simulink model "HDVSim_Hybrid_Truck_Platooning"  (R2018b)
settings: Solver=ode3  StartTime=0.0  StopTime=inf  FixedStep=sample_time  MaxStep=0.1  RelTol=1e-3  EnableMultiTasking=on
model workspace (MAT data in the model file):
  Anschaffungskosten = [3707764736; 2; 1; 1; 1; 1]
  Bat.SOC_start = 1
  Bat.Voltage = 800
  Bat.Useable_range = 0.8
  Bat.Charge_cycles = 3202.25561185
  Bat.Useable_capacity = 61.538
  Bat.Efficiency_power_electronics = 0.95
  Bat.Type = 2
  Driving_cycle = 18
  Eigenschaften = []
  Electric_Truck = 0
  Elektro_LKW = 0
  FuelCell.P_nom = 0
  Fueltype = 1
  Gewichte = [3707764736; 2; 1; 1; 2; 2]
  Hybrid_Truck = 0
  IZ12 = 3600
  Kraftstoff = 1
  M_el = 1000
  SOC_T_EM_completely_available = 0.5
  SOC_addition = 0.4
  SOC_el = 0.8
  SOC_target = 0.85
  Sailing_without_drag_torque = 0
  TCO = TCO
  TCO.Verhaeltnis_Anh_Lkw = [1 1]
  TCO.Kaufpreis = [89248 59191]
  TCO.Preisanstieg_Wiederbeschaffung = [3.5 3.5]
  TCO.Wiederbeschaffungsneupreis = [59774 54183]
  TCO.Restwert = [26774 0]
  TCO.CNG_Verbrauch = 0
  TCO.LNG_Verbrauch = 0
  TCO.Wasserstoffverbrauch = 0
  TCO.Reifenkosten_Satz = [2700 5008]
  TCO.Abschreibungswert = [73478 81874]
  TCO.Mautsatz = 0.135
  TCO.Tagesarbeitszeit = 8
  TCO.Sonstige_Arbeiten_Tag = 0.5
  TCO.Bruttostundenlohn_Fahrer = 13
  TCO.Einsatztage_Jahr = 240
  TCO.Jahresbruttolohn_Fahrer = 24960
  TCO.Personalfaktor = 1.3
  TCO.Jahresbruttolohn_FZG = 32448
  TCO.Sozialaufwendungen_Proz = 25.75
  TCO.Sozialaufwendungen_EUR = 8355
  TCO.Aushilfsfahrer = 0
  TCO.Spesen_Tag = 12
  TCO.Spesen_Jahr = 2880
  TCO.Fahrerkosten_Sonstige = 0
  TCO.Fahrpersonalkosten_Summe = 43683
  TCO.Dieselpreis = 0.95
  TCO.Dieselpreis_Fremd = 1
  TCO.Adbluepreis = 0.68
  TCO.CNGpreis = 0.88
  TCO.LNGpreis = 0.81
  TCO.Strompreis = 0.12
  TCO.Wasserstoffpreis = 9
  TCO.Verzinsung_Umlaufvermoegen = 8.4
  TCO.Verzinsung_Anlagevermoegen = 8.4
  TCO.Verwaltungskosten = 10.7
  TCO.Fahrtstrecke = 50.1189193262
  TCO.Anteil_Mautstrecke = 75
  TCO.Beladezeit_Gespann = 0.25
  TCO.Entladezeit_Gespann = 0.25
  TCO.Anteil_Leerfahrten = 0
  TCO.Durchschnittsgeschwindigkeit = 84.1549018536
  TCO.Tageslenkzeit = 4.08
  TCO.Jahresfahrleistung = [82404 82404]
  TCO.Nutzungsdauer = [6 12]
  TCO.Reifenfahrleistung = [140000 170000]
  TCO.Anteil_Eigentankung_Diesel = 75
  TCO.Schmierstoffverbauch = 1
  TCO.Adblueverbrauch = 4
  TCO.Afa_zeitabhaengig = [100 100]
  TCO.Afa_leistungsabhaengig = [0 0]
  TCO.Umlaufvermoegen = [6000 1400]
  TCO.Steuern = [556 373]
  TCO.Versicherung_Kfz = [6298 677]
  TCO.Versicherung_Transport = 1000
  TCO.Kommunikation = 600
  TCO.Reparaturen_Wartung_Pflege = [0.13 0.025]
  TCO.Abschreibung_zeitabh = [12246 6823]
  TCO.Umlaufvermoegen_verzinst = 622
  TCO.Anlagevermoegen_verzinst = [3748 2486]
  TCO.Versicherung = [7298 677]
  TCO.Summe_Fzg_Kosten = [25070 10359]
  TCO.Summe_fixe_Kosten = [68753 10359]
  TCO.Abschreibung_leistungsabh = [0 0]
  TCO.Reparaturkosten = [10713 2060]
  TCO.Reifenkosten = [1589 2428]
  TCO.Lebensdauer_Batteriepack = 0
  TCO.Anschaffungspreis_Akkupack = 0
  TCO.Verschleisskosten_Batteriepack = 0
  TCO.Summe_variable_Kosten = [12302 4488]
  TCO.Summe_fixe_variable_Kosten = [81055 14847]
  TCO.Gemeinkosten = 11491
  TCO.Mautkosten = 8343.405
  TCO.Gesamtkosten = 115736.405
  TCO.Ergebnis = table
  TCO.Ergebnis.data = {{[]; 19069; 622; 6234; 929; 7975; 600; 35429; 43683; 79112; []; 0; 0; 0; 12773; 0; 4017; 16790; []; 95902; 11491; 8343.405; 115736.405}, {[]; 0.231408669482; 0.00754817727295; 0.0756516673948; 0.0112737245765; 0.0967792825591; 0.00728119994175; 0.429942721227; 0.530107761759; 0.960050482986; []; 0; 0; 0; 0.155004611427; 0; 0.04874763361; 0.203752245037; []; 1.16380272802; 0.139447114218; 0.10125; 1.40449984224}, {[]; []; []; []; []; []; []; []; []; []; []; []; []; []; []; []; []; []; []; []; []; []; []}, {'#cccccc'; '#9DFF00'; '#CEFF00'; '#FFFF00'; '#FFDF00'; '#FFB900'; '#FF9200'; '#FF5D00'; '#FF7F7F'; '#FF2900'; '#cccccc'; '#00FF85'; '#00FFC6'; '#00FFF2'; '#00FFFF'; '#00DBFF'; '#00B3FF'; '#0088FF'; '#cccccc'; '#B100FF'; '#FF00FF'; '#FF00C0'; '#FF0070'}, [0; 1; 1; 1; 1; 1; 1; 0; 1; 0; 0; 1; 1; 1; 1; 1; 1; 0; 0; 0; 1; 1; 0]}
  TCO.Ergebnis.ndims = 2
  TCO.Ergebnis.nrows = 23
  TCO.Ergebnis.rownames = {'Zeitabh_Fzg_Kosten'; 'Abschreibung_zeitabh'; 'Umlaufvermoegen_verzinst'; 'Anlagevermoegen_verzinst'; 'Steuern'; 'Versicherung'; 'Kommunikation'; 'Summe_Fzg_Kosten'; 'Fahrpersonalkosten_Summe'; 'Summe_fixe_Kosten'; 'Leistungsabh_Fzg_Kosten'; 'Abschreibung_leistungsabh'; 'Kraftstoffkosten'; 'Adbluekosten'; 'Reparaturkosten'; 'Schmierstoffkosten'; 'Reifenkosten'; 'Summe_variable_Kosten'; 'Summe_Kosten'; 'Summe_fixe_variable_Kosten'; 'Gemeinkosten'; 'Mautkosten'; 'Gesamtkosten'}
  TCO.Ergebnis.nvars = 5
  TCO.Ergebnis.varnames = {'Euro_Jahr', 'Euro_km', 'Prozent', 'Cellcolor', 'Diagramm'}
  TCO.Ergebnis.props.CustomProps = struct()
  TCO.Ergebnis.props.VariableCustomProps = struct()
  TCO.Ergebnis.props.versionSavedFrom = 3
  TCO.Ergebnis.props.minCompatibleVersion = 1
  TCO.Ergebnis.props.incompatibilityMsg = ''
  TCO.Ergebnis.props.VersionSavedFrom = 3
  TCO.Ergebnis.props.Description = ''
  TCO.Ergebnis.props.DimensionNames = {'Row', 'Variables'}
  TCO.Ergebnis.props.UserData = []
  TCO.Ergebnis.props.VariableDescriptions = {}
  TCO.Ergebnis.props.VariableUnits = {}
  TCO.Ergebnis.props.VariableContinuity = {}
  TCO_Anhaenger = 1
  TCO_Trailer = 1
  T_distance_LPS_down = 250
  T_distance_LPS_up = 250
  VSim.Display = 3
  VSim.Opt = 0
  VSim.v_t = [0 0 0 0 0 0 1.65166299447 3.48693546103 5.32196202623 7.15649366725 8.99043956604 10.9164984764 14.0784276146 19.1118285963 24.3934691092 29.026743167 31.4408667289 30.4086481328 33.8215646226 37.2573263956 40.6862952223 44.1078751777 47.5214696449 50.9264939062 54.3223705164 57.7085257373 61.0843888586 64.4493705574 67.8028976245 71.1444114206 74.4733381735 77.7891152098 81.0911158753 84.3786820499 87.3671173407 86.464344428 86.4690301672 86.4747021938 86.4803197388 86.4858626831 86.4913275703 86.4967182207 86.5020271743]
  Vehicle = 'empty'
  WPT.Voltage = 0
  WPT.P_max = 120
  WPT.expansion = 0.42
  WPT.eta = 0.92
  WPT.SOC_target = 1
  WPT.SOC_electric_only = 1
  acquisition_costs = [3707764736; 2; 1; 1; 5; 5]
  addition_for_critical_slope = 0.01
  ambient.gravity = 9.80665
  ambient.air_density = 1.1883
  ambient.friction_coeff = 0.8
  auxiliary_consumers.onBattery = 0
  auxiliary_consumers.power = 3500
  auxiliary_consumers.coolingSystem = [2.07882285003 1.39429153551 1.17315152225 1.09571031996 1.06766795776 1.05740509167 1.05341861849 1.05184466719 1.05110543918 1.05094477446 1.05078585401 1.05075614757 ... (2400 elements, 2400x1)]
  critical_altitude_difference = 50
  cycle.stop_end = 5
  cycle.stop_start = 5
  cycle.speed_init = 0
  cycle.distance = [1 2 3 4 5 6 7 8 9 10 11 12 ... (50000 elements, 1x50000)]
  cycle.speed = [23.6111111111 23.6111111111 23.6111111111 23.6111111111 23.6111111111 23.6111111111 23.6111111111 23.6111111111 23.6111111111 23.6111111111 23.6111111111 23.6111111111 ... (50000 elements, 1x50000)]
  cycle.slope = [-0.005 -0.005 -0.005 -0.005 -0.005 -0.005 -0.005 -0.005 -0.005 -0.005 -0.005 -0.005 ... (50000 elements, 1x50000)]
  cycle.altitude = [0 0 0 0 0 0 0 0 0 0 0 0 ... (50000 elements, 1x50000)]
  cycle.delta12 = [5 5 5 5 5 5 5 5 5 5 5 5 ... (50000 elements, 1x50000)]
  cycle.delta23 = [5 5 5 5 5 5 5 5 5 5 5 5 ... (50000 elements, 1x50000)]
  cycle.stop_time = [0 0 0 0 0 0 0 0 0 0 0 0 ... (50000 elements, 1x50000)]
  dcycle = 18
  distance_1_PPC = 175
  distance_2_PPC = 200
  distance_PPC_altitude_difference = 10000
  driver.controller_proportional_gain = 230000
  driver.controller_integral_gain = 3000
  driver.slew_rate_throttle_in = 2
  driver.slew_rate_throttle_out = -2
  driver.slew_rate_brake_in = 2
  driver.slew_rate_brake_out = -2
  em.P_max = 130
  em.M_max = 1050
  em.n_max = 2000
  em.n_eck = 1182.29386297
  em.speed = [0 10 20 30 40 50 60 70 80 90 100 110 120 130 140 150 160 170 180 190 200 210 220 230 240 250 260 270 280 290 300 310 320 330 340 350 360 370 380 390 400 410 420 430 440 450 460 470 480 490 500 510 520 530 540 550 560 570 580 590 600 610 620 630 640 650 660 670 680 690 700 710 720 730 740 750 760 770 780 790 800 810 820 830 840 850 860 870 880 890 900 910 920 930 940 950 960 970 980 990 1000 1010 1020 1030 1040 1050 1060 1070 1080 1090 1100 1110 1120 1130 1140 1150 1160 1170 1180 1190 1200 1210 1220 1230 1240 1250 1260 1270 1280 1290 1300 1310 1320 1330 1340 1350 1360 1370 1380 1390 1400 1410 1420 1430 1440 1450 1460 1470 1480 1490 1500 1510 1520 1530 1540 1550 1560 1570 1580 1590 1600 1610 1620 1630 1640 1650 1660 1670 1680 1690 1700 1710 1720 1730 1740 1750 1760 1770 1780 1790 1800 1810 1820 1830 1840 1850 1860 1870 1880 1890 1900 1910 1920 1930 1940 1950 1960 1970 1980 1990 2000]
  em.trq = [1050 1050 1050 1050 1050 1050 1050 1050 1050 1050 1050 1050 1050 1050 1050 1050 1050 1050 1050 1050 1050 1050 1050 1050 1050 1050 1050 1050 1050 1050 1050 1050 1050 1050 1050 1050 1050 1050 1050 1050 1050 1050 1050 1050 1050 1050 1050 1050 1050 1050 1050 1050 1050 1050 1050 1050 1050 1050 1050 1050 1050 1050 1050 1050 1050 1050 1050 1050 1050 1050 1050 1050 1050 1050 1050 1050 1050 1050 1050 1050 1050 1050 1050 1050 1050 1050 1050 1050 1050 1050 1050 1050 1050 1050 1050 1050 1050 1050 1050 1050 1050 1050 1050 1050 1050 1050 1050 1050 1050 1050 1050 1050 1050 1050 1050 1050 1050 1050 1050 1043.20046733 1034.5071301 1025.95748439 1017.54799682 1009.27524888 1001.13593235 993.126844893 985.244885807 977.48705206 969.850434466 962.332214044 954.929658551 947.640119173 940.461027361 933.389891817 926.42429561 919.56189342 912.800408909 906.137632202 899.571417476 893.09968066 886.720397226 880.431600083 874.231377547 868.11787141 862.089275081 856.143831805 850.279832957 844.495616406 838.789564944 833.160104776 827.605704078 822.124871601 816.71615534 811.378141253 806.109452024 800.908745882 795.774715459 790.706086699 785.701617795 780.760098187 775.880347573 771.061214979 766.30157785 761.600341176 756.956436657 752.368821889 747.836479588 743.358416836 738.933664355 734.561275809 730.240327128 725.969915858 721.749160533 717.577200068 713.453193171 709.376317781 705.345770521 701.360766168 697.420537144 693.524333026 689.671420065 685.861080728 682.092613251 678.365331211 674.678563107 671.031651955 667.423954901 663.854842843 660.323700062 656.829923871 653.372924272 649.952123621 646.566956311 643.216868454 639.901317586 636.619772368 633.371712304 630.15662747 626.974018241 623.823395034 620.704278058]
  em.Type = 1
  em.fuel.co2_per_kwh = 504
  em.efficiency.characteristic_map = [0.001 0.001 0.001 0.001 0.001 0.001 0.001 0.001 0.001 0.001 0.001 0.001 ... (20301 elements, 101x201)]
  em.efficiency.speed = [0 10 20 30 40 50 60 70 80 90 100 110 120 130 140 150 160 170 180 190 200 210 220 230 240 250 260 270 280 290 300 310 320 330 340 350 360 370 380 390 400 410 420 430 440 450 460 470 480 490 500 510 520 530 540 550 560 570 580 590 600 610 620 630 640 650 660 670 680 690 700 710 720 730 740 750 760 770 780 790 800 810 820 830 840 850 860 870 880 890 900 910 920 930 940 950 960 970 980 990 1000 1010 1020 1030 1040 1050 1060 1070 1080 1090 1100 1110 1120 1130 1140 1150 1160 1170 1180 1190 1200 1210 1220 1230 1240 1250 1260 1270 1280 1290 1300 1310 1320 1330 1340 1350 1360 1370 1380 1390 1400 1410 1420 1430 1440 1450 1460 1470 1480 1490 1500 1510 1520 1530 1540 1550 1560 1570 1580 1590 1600 1610 1620 1630 1640 1650 1660 1670 1680 1690 1700 1710 1720 1730 1740 1750 1760 1770 1780 1790 1800 1810 1820 1830 1840 1850 1860 1870 1880 1890 1900 1910 1920 1930 1940 1950 1960 1970 1980 1990 2000]
  em.efficiency.torque = [0 10.5 21 31.5 42 52.5 63 73.5 84 94.5 105 115.5 126 136.5 147 157.5 168 178.5 189 199.5 210 220.5 231 241.5 252 262.5 273 283.5 294 304.5 315 325.5 336 346.5 357 367.5 378 388.5 399 409.5 420 430.5 441 451.5 462 472.5 483 493.5 504 514.5 525 535.5 546 556.5 567 577.5 588 598.5 609 619.5 630 640.5 651 661.5 672 682.5 693 703.5 714 724.5 735 745.5 756 766.5 777 787.5 798 808.5 819 829.5 840 850.5 861 871.5 882 892.5 903 913.5 924 934.5 945 955.5 966 976.5 987 997.5 1008 1018.5 1029 1039.5 1050]
  em_M_max = 1050
  engine.bsfc.be = [1463.81124945 1337.51367643 1219.93532707 1127.30261663 1034.66990619 942.037195751 849.40448531 756.771774869 664.139064428 571.506353987 478.873643547 386.240933106 ... (45451 elements, 301x151)]
  engine.bsfc.trqorig = [0 10 20 30 40 50 60 70 80 90 100 110 120 130 140 150 160 170 180 190 200 210 220 230 240 250 260 270 280 290 300 310 320 330 340 350 360 370 380 390 400 410 420 430 440 450 460 470 480 490 500 510 520 530 540 550 560 570 580 590 600 610 620 630 640 650 660 670 680 690 700 710 720 730 740 750 760 770 780 790 800 810 820 830 840 850 860 870 880 890 900 910 920 930 940 950 960 970 980 990 1000 1010 1020 1030 1040 1050 1060 1070 1080 1090 1100 1110 1120 1130 1140 1150 1160 1170 1180 1190 1200 1210 1220 1230 1240 1250 1260 1270 1280 1290 1300 1310 1320 1330 1340 1350 1360 1370 1380 1390 1400 1410 1420 1430 1440 1450 1460 1470 1480 1490 1500 1510 1520 1530 1540 1550 1560 1570 1580 1590 1600 1610 1620 1630 1640 1650 1660 1670 1680 1690 1700 1710 1720 1730 1740 1750 1760 1770 1780 1790 1800 1810 1820 1830 1840 1850 1860 1870 1880 1890 1900 1910 1920 1930 1940 1950 1960 1970 1980 1990 2000 2010 2020 2030 2040 2050 2060 2070 2080 2090 2100 2110 2120 2130 2140 2150 2160 2170 2180 2190 2200 2210 2220 2230 2240 2250 2260 2270 2280 2290 2300 2310 2320 2330 2340 2350 2360 2370 2380 2390 2400 2410 2420 2430 2440 2450 2460 2470 2480 2490 2500 2510 2520 2530 2540 2550 2560 2570 2580 2590 2600 2610 2620 2630 2640 2650 2660 2670 2680 2690 2700 2710 2720 2730 2740 2750 2760 2770 2780 2790 2800 2810 2820 2830 2840 2850 2860 2870 2880 2890 2900 2910 2920 2930 2940 2950 2960 2970 2980 2990 3000]
  engine.bsfc.speed = [600 610 620 630 640 650 660 670 680 690 700 710 720 730 740 750 760 770 780 790 800 810 820 830 840 850 860 870 880 890 900 910 920 930 940 950 960 970 980 990 1000 1010 1020 1030 1040 1050 1060 1070 1080 1090 1100 1110 1120 1130 1140 1150 1160 1170 1180 1190 1200 1210 1220 1230 1240 1250 1260 1270 1280 1290 1300 1310 1320 1330 1340 1350 1360 1370 1380 1390 1400 1410 1420 1430 1440 1450 1460 1470 1480 1490 1500 1510 1520 1530 1540 1550 1560 1570 1580 1590 1600 1610 1620 1630 1640 1650 1660 1670 1680 1690 1700 1710 1720 1730 1740 1750 1760 1770 1780 1790 1800 1810 1820 1830 1840 1850 1860 1870 1880 1890 1900 1910 1920 1930 1940 1950 1960 1970 1980 1990 2000 2010 2020 2030 2040 2050 2060 2070 2080 2090 2100]
  engine.bsfc.M_be_min_orig = [1000 1040 1080 1120 1130 1140 1150 1160 1170 1180 1190 1200 1480 1520 1560 1600 1640 1680 1720 1760 1800 1840 1880 1920 1960 2000 2040 2080 2120 2160 2200 2220 2240 2240 2240 2240 2230 2230 2140 2130 2130 2130 2130 2130 2130 2130 2130 2030 1840 1840 1830 1830 1830 1830 1830 1830 1830 1830 1830 1730 1730 1730 1730 1730 1720 1720 1720 1720 1720 1720 1720 1720 1720 1720 1720 1720 1720 1720 1720 1720 1710 1720 1710 1710 1710 1620 1620 1620 1620 1620 1620 1630 1640 1640 1650 1660 1670 1680 1690 1700 1710 1710 1710 1710 1710 1710 1710 1710 1710 1710 1900 1890 1890 1890 1890 1890 1890 1890 1880 1870 1860 1840 1830 1820 1810 1800 1780 1770 1760 1750 1740 1720 1710 1700 1690 1680 1660 1650 1640 1630 1620 0 0 0 0 0 0 0 0 0 0]
  engine.bsfc.trq = [0 10 20 30 40 50 60 70 80 90 100 110 120 130 140 150 160 170 180 190 200 210 220 230 240 250 260 270 280 290 300 310 320 330 340 350 360 370 380 390 400 410 420 430 440 450 460 470 480 490 500 510 520 530 540 550 560 570 580 590 600 610 620 630 640 650 660 670 680 690 700 710 720 730 740 750 760 770 780 790 800 810 820 830 840 850 860 870 880 890 900 910 920 930 940 950 960 970 980 990 1000 1010 1020 1030 1040 1050 1060 1070 1080 1090 1100 1110 1120 1130 1140 1150 1160 1170 1180 1190 1200 1210 1220 1230 1240 1250 1260 1270 1280 1290 1300 1310 1320 1330 1340 1350 1360 1370 1380 1390 1400 1410 1420 1430 1440 1450 1460 1470 1480 1490 1500 1510 1520 1530 1540 1550 1560 1570 1580 1590 1600 1610 1620 1630 1640 1650 1660 1670 1680 1690 1700 1710 1720 1730 1740 1750 1760 1770 1780 1790 1800 1810 1820 1830 1840 1850 1860 1870 1880 1890 1900 1910 1920 1930 1940 1950 1960 1970 1980 1990 2000 2010 2020 2030 2040 2050 2060 2070 2080 2090 2100 2110 2120 2130 2140 2150 2160 2170 2180 2190 2200 2210 2220 2230 2240 2250 2260 2270 2280 2290 2300 2310 2320 2330 2340 2350 2360 2370 2380 2390 2400 2410 2420 2430 2440 2450 2460 2470 2480 2490 2500 2510 2520 2530 2540 2550 2560 2570 2580 2590 2600 2610 2620 2630 2640 2650 2660 2670 2680 2690 2700 2710 2720 2730 2740 2750 2760 2770 2780 2790 2800 2810 2820 2830 2840 2850 2860 2870 2880 2890 2900 2910 2920 2930 2940 2950 2960 2970 2980 2990 3000]
  engine.bsfc.M_be_min = [1000 1040 1080 1120 1130 1140 1150 1160 1170 1180 1190 1200 1480 1520 1560 1600 1640 1680 1720 1760 1800 1840 1880 1920 1960 2000 2040 2080 2120 2160 2200 2220 2240 2240 2240 2240 2230 2230 2140 2130 2130 2130 2130 2130 2130 2130 2130 2030 1840 1840 1830 1830 1830 1830 1830 1830 1830 1830 1830 1730 1730 1730 1730 1730 1720 1720 1720 1720 1720 1720 1720 1720 1720 1720 1720 1720 1720 1720 1720 1720 1710 1720 1710 1710 1710 1620 1620 1620 1620 1620 1620 1630 1640 1640 1650 1660 1670 1680 1690 1700 1710 1710 1710 1710 1710 1710 1710 1710 1710 1710 1900 1890 1890 1890 1890 1890 1890 1890 1880 1870 1860 1840 1830 1820 1810 1800 1780 1770 1760 1750 1740 1720 1710 1700 1690 1680 1660 1650 1640 1630 1620 0 0 0 0 0 0 0 0 0 0]
  engine.full_load.speed = [600; 900; 1000; 1350; 2000; 2001; 2100]
  engine.full_load.trqorig = [1000; 2200; 2400; 2400; 1620; 0; 0]
  engine.full_load.trq = [1000; 2200; 2400; 2400; 1620; 0; 0]
  engine.full_load.power = [62.8318530718; 207.345115137; 251.327412287; 339.292006588; 339.292006588; 0; 0]
  engine.number = 1
  engine.M_max_original = 2400
  engine.M_max = 2400
  engine.scale_factor = 1
  engine.fuel.density = 830
  engine.fuel.co2_per_litre = 2.62
  engine.fuel.heat_of_combustion = 42500
  engine.fuel.LHV = 35.8
  engine.speed_min = 600
  engine.speed_max = 2100
  engine.idle_fuel_consumption = 1.5
  engine.drag_torque.trq = [0 -65.6 -98.9 -123.3 -134.32 -156.04 -176.72 -217.28 -234.63 -256.02 -273.98 -301.74 -324 -353.92 -376.32 -421.26 -450]
  engine.drag_torque.speed = [0 450 600 700 800 1000 1200 1500 1600 1700 1800 1900 2000 2100 2200 2300 2400]
  engine.rated_power = 323619.35891
  engine.shift_parameter.n_lo = 1000
  engine.shift_parameter.n_pref = 1200
  engine.shift_parameter.n1 = 600
  engine.shift_parameter.n2 = 800
  engine.shift_parameter.n3 = 1100
  engine.shift_parameter.n4 = 600
  engine.shift_parameter.n5 = 1200
  engine.shift_parameter.n6 = 2100
  engine.shift_parameter.M_max = 2400
  final_drive.ratio = 10
  final_drive.trq_eff = 0.98
  ifElectric = 1
  ifOptimized = 0
  look_ahead_PPC = 250
  max_distance = 50000
  name = 'Verbrauchssimulation_Hybrid_LKW_Platooning'
  propertie = [3707764736; 2; 1; 1; 6; 6]
  prospective_cruise_control = 0
  sample_time = 0.1
  tank.v_diesel = 500
  tank.v_cng = 0
  tank.v_lng = 0
  tank.m_h2 = 0
  tires.radius = 0.4465
  tires.roll_drag_coeff.total = 0.0043
  transmission.init_gear = 1
  transmission.shift_time = 1
  transmission.ratios = [1 1]
  transmission.trq_eff = [0.99 0.99]
  transmission.lamda = [1.0130058518 1.0130058518]
  transmission.z = 1
  v_PPC_delta = 2.77777777778
  v_max_electrical_drive_only = 13.8888888889
  vehicle.long_truck = 0
  vehicle.payload = 19300
  vehicle.frontal_area = 10.2
  vehicle.air_drag_coeff = [0.527  0.527  0.527  0.527  0.527  0.527  0.527  0.527  0.527  0.527; 0.527  0.527  0.527  0.527  0.527  0.527  0.527  0.527  0.527  0.527; 0.527  0.527  0.527  0.527  0.527  0.527  0.527  0.527  0.527  0.527; 0.527  0.527  0.527  0.527  0.527  0.527  0.527  0.527  0.527  0.527; 0.527  0.527  0.527  0.527  0.527  0.527  0.527  0.527  0.527  0.527; 0.527  0.527  0.527  0.527  0.527  0.527  0.527  0.527  0.527  0.527; 0.527  0.527  0.527  0.527  0.527  0.527  0.527  0.527  0.527  0.527; 0.527  0.527  0.527  0.527  0.527  0.527  0.527  0.527  0.527  0.527; 0.527  0.527  0.527  0.527  0.527  0.527  0.527  0.527  0.527  0.527; 0.527  0.527  0.527  0.527  0.527  0.527  0.527  0.527  0.527  0.527]
  vehicle.Fx_max = 90221.18
  vehicle.F_brake_max = 309890.14
  vehicle.mass = 12632.5464604
  vehicle_F_brake_max = 309890.14
  weights = weights
  weights.m_Engine = 1122.29
  weights.m_Gearbox = 125
  weights.m_Retarder = 82
  weights.m_tank_system = 51.6564603608
  weights.m_Fuel = 425
  weights.m_Exhaust = 203.4
  weights.m_Trailer = 5400
  weights.m_Total = 7232.54646036
  weights.m_Base = 5223.2
  weights.max_Payload = 27367.4535396
  weights.m_Max = 40000
  x = 1
values from neighbouring files (symbols this model uses):
  transmission = Transmission_gearing(1, 1, false, false, final_drive.ratio)    [Parameterizing.m]
undefined symbols (not defined in the file or in its folder): Ion, Lithium
libraries: simulink x23, powerlib x2, electricdrivelib x1
(part 1 of 3)
settings Model: Creator=Alexander Suessmann  LastModifiedBy=ga73rep
settings DataIOCC: SaveFormat=Array  SaveOutput=off  SignalLogging=off  DSMLogging=off  SignalLoggingName=datalog
settings OptimizationCC: DefaultParameterBehavior=Inlined  ExpressionDepthLimit=2147483647  InitFltsAndDblsToZero=on  LifeSpan=inf
settings DebuggingCC: UnderspecifiedInitializationDetection=Classic  MergeDetectMultiDrivingBlocksExec=none  SolverPrmCheckMsg=warning  MultiTaskDSMMsg=warning  MultiTaskCondExecSysMsg=none  FcnCallInpInsideContextMsg=warning  AllowSymbolicDim=off  StateNameClashWarn=warning  SFUnusedDataAndEventsDiag=none  SFUnexpectedBacktrackingDiag=none  SFInvalidInputDataAccessInChartInitDiag=none  SFNoUnconditionalDefaultTransitionDiag=none  SFTransitionOutsideNaturalParentDiag=none  SFUnreachableExecutionPathDiag=none  SFUndirectedBroadcastEventsDiag=none  SFTransitionActionBeforeConditionDiag=none  SFExecutionAtInitializationDiag=none
settings HardwareCC: ProdBitPerPointer=32  ProdBitPerSizeT=32  ProdBitPerPtrDiffT=32  ProdLargestAtomicFloat=None  ProdIntDivRoundTo=Undefined  ProdEndianess=Unspecified  ProdWordSize=32  ProdHWDeviceType=32-bit Generic
settings ModelReferenceCC: PropagateSignalLabelsOutOfModel=off
settings SFSimCC: SimUseLocalCustomCode=off
settings RTWCC: RTWUseLocalCustomCode=off
settings CodeAppCC: StateflowObjectComments=on
settings GRTTargetCC: TargetLangStandard=C89/C90 (ANSI)  GeneratePreprocessorConditionals=Disable all  CombineOutputUpdateFcns=off  GRTInterface=on
settings ConfigComp: CovMetricSettings=dw  CovHtmlReporting=on  CovSaveCumulativeToWorkspaceVar=on  CovSaveSingleToWorkspaceVar=on  CovExternalEMLEnable=off  CovSFcnEnable=off
settings SimscapeCC: SimscapeNormalizeSystem=off

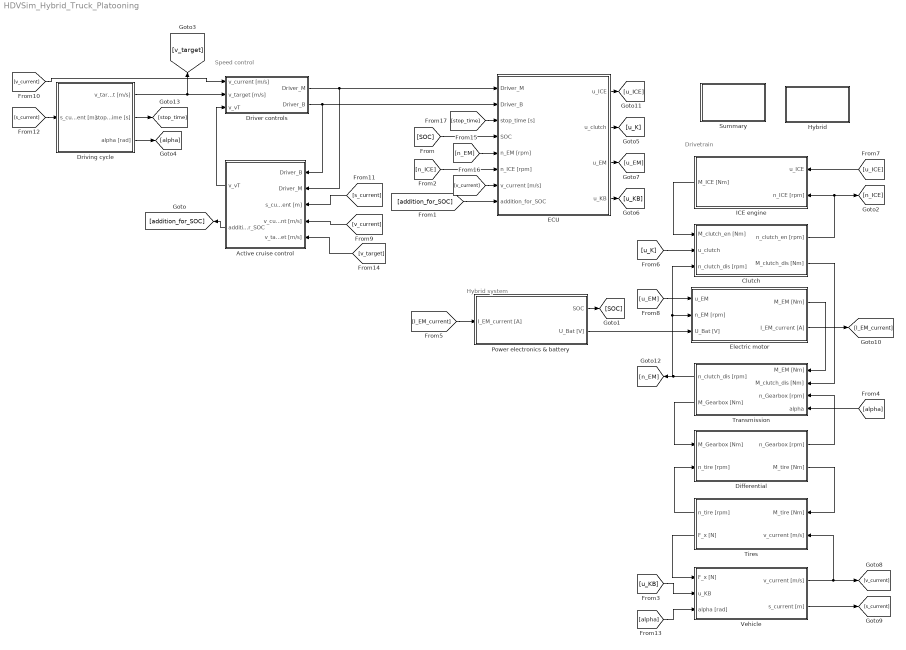
== system HDVSim_Hybrid_Truck_Platooning ==
  note: Hybrid system
  note: Speed control
  note: Drivetrain
  Active cruise control : Subsystem
  Clutch : Subsystem
  Differential : Subsystem
  Driver controls : Subsystem
  Driving cycle : Subsystem
  ECU : Subsystem
  Electric motor : Subsystem
  Hybrid : Subsystem
  ICE engine : Subsystem
  Power electronics & battery : Subsystem
  Summary : Subsystem
  Tires : Subsystem
  Transmission : Subsystem
  Vehicle : Subsystem
  wires:
  ICE engine/1(M_ICE [Nm]) -> Clutch/1(M_clutch_en [Nm])
  Transmission/1(n_clutch_dis [rpm]) -> Clutch/3(n_clutch_dis [rpm]), Electric motor/2(n_EM [rpm]), [n_EM]
  Transmission/2(M_Gearbox [Nm]) -> Differential/1(M_Gearbox [Nm])
  Tires/1(n_tire [rpm]) -> Differential/2(n_tire [rpm])
  Clutch/1(n_clutch_en [rpm]) -> [n_ICE], ICE engine/2(n_ICE [rpm])
  Clutch/2(M_clutch_dis [Nm]) -> Transmission/2(M_clutch_dis [Nm])
  Differential/1(n_Gearbox [rpm]) -> Transmission/3(n_Gearbox [rpm])
  Differential/2(M_tire [Nm]) -> Tires/1(M_tire [Nm])
  Vehicle/1(v_current [m/s]) -> [v_current], Tires/2(v_current [m/s])
  Tires/2(F_x [N]) -> Vehicle/1(F_x [N])
  Driver controls/2(Driver_B) -> Active cruise control/1(Driver_B), ECU/2(Driver_B)
  Electric motor/1(M_EM [Nm]) -> Transmission/1(M_EM [Nm])
  Active cruise control/2(addition_for_SOC) -> [addition_for_SOC]
  [addition_for_SOC] -> ECU/8(addition_for_SOC)
  Power electronics & battery/1(SOC) -> [SOC]
  [SOC] -> ECU/4(SOC)
  [n_ICE] -> ECU/6(n_ICE [rpm])
  Driving cycle/1(v_target [m/s]) -> [v_target], Driver controls/2(v_target [m/s])
  [v_current] -> Driver controls/1(v_current [m/s])
  [s_current] -> Driving cycle/1(s_current [m])
  Driving cycle/3(alpha [rad]) -> [alpha]
  Active cruise control/1(v_vT) -> Driver controls/3(v_vT)
  Driver controls/1(Driver_M) -> Active cruise control/2(Driver_M), ECU/1(Driver_M)
  [s_current] -> Active cruise control/3(s_current [m])
  [v_current] -> Active cruise control/4(v_current [m/s])
  [v_target] -> Active cruise control/5(v_target [m/s])
  Power electronics & battery/2(U_Bat [V]) -> Electric motor/3(U_Bat [V])
  [u_EM] -> Electric motor/1(u_EM)
  ECU/2(u_clutch) -> [u_K]
  [u_K] -> Clutch/2(u_clutch)
  ECU/4(u_KB) -> [u_KB]
  [u_KB] -> Vehicle/2(u_KB)
  [alpha] -> Vehicle/3(alpha [rad])
  Vehicle/2(s_current [m]) -> [s_current]
  [alpha] -> Transmission/4(alpha)
  Electric motor/2(I_EM_current [A]) -> [I_EM_current]
  [I_EM_current] -> Power electronics & battery/1(I_EM_current [A])
  ECU/3(u_EM) -> [u_EM]
  ECU/1(u_ICE) -> [u_ICE]
  [u_ICE] -> ICE engine/1(u_ICE)
  [n_EM] -> ECU/5(n_EM [rpm])
  [v_current] -> ECU/7(v_current [m/s])
  Driving cycle/2(stop_time [s]) -> [stop_time]
  [stop_time] -> ECU/3(stop_time [s])

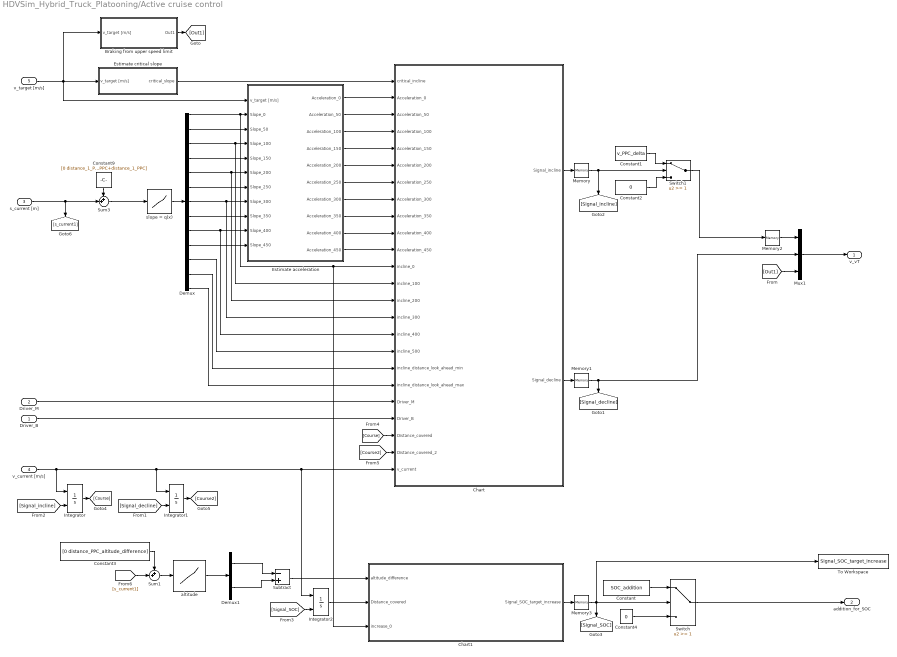
== system HDVSim_Hybrid_Truck_Platooning/Active cruise control ==
  Driver_B : Inport
  Driver_M : Inport  Port=2
  s_current [m] : Inport  Port=3
  v_current [m/s] : Inport  Port=4
  v_target [m/s] : Inport  Port=5
  Braking from upper speed limit : Subsystem
  Chart : Stateflow chart  TreatAsAtomicUnit=on
  Chart1 : Stateflow chart  TreatAsAtomicUnit=on
  Constant : Constant  Value=SOC_addition
  Constant1 : Constant  Value=v_PPC_delta
  Constant2 : Constant  Value=0
  Constant3 : Constant  Value=[0 distance_PPC_altitude_difference]
  Constant4 : Constant  Value=0
  Constant9 : Constant  Value=[0 distance_1_PPC/5 2*distance_1_PPC/5 3*distance_1_PPC/5 4*distance_1_PPC/5 distance_1_PPC 6*distance_1_PPC/5 7*distance_1_PPC/5 8*distance_1_PPC/5 9*distance_1_PPC/5 10*distance_1_PPC/5 look_ahead_PPC look_ahead_PPC+distance_1_PPC]
  Demux : Demux  Outputs=13
  Demux1 : Demux  Outputs=2
  Estimate acceleration : Subsystem
  Estimate critical slope : Subsystem
  Integrator : Integrator  ExternalReset=rising
  Integrator1 : Integrator  ExternalReset=rising
  Integrator2 : Integrator  ExternalReset=rising
  Memory{,1..3} (4 alike) : Memory
  Mux1 : Mux  Inputs=3
  Subtract : Sum  Inputs=-+
  Sum1 : Sum  Inputs=++|
  Sum3 : Sum  Inputs=++|
  Switch : Switch  Threshold=1
  Switch1 : Switch  Threshold=1
  To Workspace : ToWorkspace  VariableName=Signal_SOC_target_increase  SaveFormat=Structure With Time  SampleTime=-1
  altitude : Lookup_n-D  NumberOfTableDimensions=1  BreakpointsForDimension1=cycle.distance  Table=cycle.altitude  InterpMethod=Flat  RndMeth=Simplest  InputSameDT=on
  slope = q(x) : Lookup  InputValues=cycle.distance  Table=cycle.slope  LookUpMeth=Interpolation-Use End Values
  v_vT : Outport
  addition_for_SOC : Outport  Port=2
  wires:
  slope = q(x)/1 -> Demux/1
  Demux/1 -> Chart1/3(increase_0), Chart/12(incline_0), Estimate acceleration/2(Slope_0)
  Estimate critical slope/1(critical_slope) -> Chart/1(critical_incline)
  Chart/1(Signal_incline) -> Memory/1
  v_current [m/s]/1 -> Integrator/1, Integrator1/1, Chart/24(v_current), Integrator2/1
  Memory/1 -> [Signal_incline], Switch1/2
  Mux1/1 -> v_vT/1
  Constant9/1 -> Sum3/1
  Sum3/1 -> slope = q(x)/1
  Estimate acceleration/1(Acceleration_0) -> Chart/2(Acceleration_0)
  Estimate acceleration/2(Acceleration_50) -> Chart/3(Acceleration_50)
  Estimate acceleration/3(Acceleration_100) -> Chart/4(Acceleration_100)
  Estimate acceleration/4(Acceleration_150) -> Chart/5(Acceleration_150)
  Estimate acceleration/5(Acceleration_200) -> Chart/6(Acceleration_200)
  Estimate acceleration/6(Acceleration_250) -> Chart/7(Acceleration_250)
  Estimate acceleration/7(Acceleration_300) -> Chart/8(Acceleration_300)
  Estimate acceleration/8(Acceleration_350) -> Chart/9(Acceleration_350)
  Chart/2(Signal_decline) -> Memory1/1
  Memory1/1 -> Mux1/2, [Signal_decline]
  Driver_B/1 -> Chart/21(Driver_B)
  Estimate acceleration/9(Acceleration_400) -> Chart/10(Acceleration_400)
  Estimate acceleration/10(Acceleration_450) -> Chart/11(Acceleration_450)
  Driver_M/1 -> Chart/20(Driver_M)
  Demux/2 -> Estimate acceleration/3(Slope_50)
  Demux/3 -> Chart/13(incline_100), Estimate acceleration/4(Slope_100)
  Demux/4 -> Estimate acceleration/5(Slope_150)
  Demux/5 -> Chart/14(incline_200), Estimate acceleration/6(Slope_200)
  Demux/6 -> Estimate acceleration/7("Slope_250 ")
  Demux/7 -> Chart/15(incline_300), Estimate acceleration/8(Slope_300)
  Demux/8 -> Estimate acceleration/9(Slope_350)
  Demux/9 -> Chart/16(incline_400), Estimate acceleration/10(Slope_400)
  Demux/10 -> Estimate acceleration/11(Slope_450)
  Demux/12 -> Chart/18(incline_distance_look_ahead_min)
  Demux/13 -> Chart/19(incline_distance_look_ahead_max)
  v_target [m/s]/1 -> Braking from upper speed limit/1(v_target [m/s]), Estimate acceleration/1(v_target [m/s]), Estimate critical slope/1(v_target [m/s])
  Memory2/1 -> Mux1/1
  Constant1/1 -> Switch1/1
  Constant2/1 -> Switch1/3
  Demux/11 -> Chart/17(incline_500)
  Switch1/1 -> Memory2/1
  Constant3/1 -> Sum1/1
  s_current [m]/1 -> [s_current1], Sum3/2
  Sum1/1 -> altitude/1
  altitude/1 -> Demux1/1
  Demux1/2 -> Subtract/2
  Demux1/1 -> Subtract/1
  Subtract/1 -> Chart1/1(altitude_difference)
  Chart1/1(Signal_SOC_target_increase) -> Memory3/1
  Integrator2/1 -> Chart1/2(Distance_covered)
  Constant/1 -> Switch/1
  Constant4/1 -> Switch/3
  Switch/1 -> addition_for_SOC/1
  Memory3/1 -> Switch/2, To Workspace/1, [Signal_SOC]
  [Signal_decline] -> Integrator1/2
  Integrator1/1 -> [Course2]
  Integrator/1 -> [Course]
  [Signal_incline] -> Integrator/2
  [Course] -> Chart/22(Distance_covered)
  [Course2] -> Chart/23(Distance_covered_2)
  [Signal_SOC] -> Integrator2/2
  [s_current1] -> Sum1/2
  Braking from upper speed limit/1(Out1) -> [Out1]
  [Out1] -> Mux1/3

== system HDVSim_Hybrid_Truck_Platooning/Clutch ==
  note: Torque where clutch is disengaged
  note: Speed where clutch is engaged
  M_clutch_en [Nm] : Inport
  u_clutch : Inport  Port=2
  n_clutch_dis [rpm] : Inport  Port=3
  Compare To Zero : simulink/Logic and Bit Operations/Compare To Zero  relop===  OutDataTypeStr=boolean
  Constant : Constant  Value=0
  Idle engine speed : Constant  Value=engine.speed_min
  Logical Operator : Logic  AllPortsSameDT=off  OutDataTypeStr=boolean
  Lower engine speed : Saturate  UpperLimit=10000  LowerLimit=engine.speed_min  ZeroCross=off
  Null1 : Constant  Value=0
  Switch1 : Switch  Threshold=1
  Switch2 : Switch  Threshold=1
  Switch3 : Switch  Threshold=1
  n_clutch_en [rpm] : Outport
  M_clutch_dis [Nm] : Outport  Port=2
  wires:
  n_clutch_dis [rpm]/1 -> Lower engine speed/1
  Lower engine speed/1 -> Switch3/3
  Switch2/1 -> Switch1/3
  Null1/1 -> Switch2/1
  M_clutch_en [Nm]/1 -> Switch2/3
  [M_mot] -> Compare To Zero/1
  Compare To Zero/1 -> Logical Operator/1
  [ZKU] -> Logical Operator/2
  Logical Operator/1 -> Switch2/2
  Switch1/1 -> M_clutch_dis [Nm]/1
  Constant/1 -> Switch1/1
  Switch3/1 -> n_clutch_en [rpm]/1
  u_clutch/1 -> Switch1/2, Switch3/2
  Idle engine speed/1 -> Switch3/1

== system HDVSim_Hybrid_Truck_Platooning/Differential ==
  note: Effective wheel torque
  M_Gearbox [Nm] : Inport
  n_tire [rpm] : Inport  Port=2
  Differential efficiency : Constant  Value=final_drive.trq_eff
  Differential gear ratio : Constant  Value=final_drive.ratio
  M' = M*i*eta : Product  Inputs=***
  Product : Product  Inputs=/  RndMeth=Zero
  Switch : Switch  ZeroCross=off
  n' *i = n : Product  RndMeth=Zero
  n_Gearbox [rpm] : Outport
  M_tire [Nm] : Outport  Port=2
  tag scope: Eta_Axle_Drive=global
  wires:
  M_Gearbox [Nm]/1 -> M' = M*i*eta/1, Switch/2
  n_tire [rpm]/1 -> n' *i = n/2
  Differential gear ratio/1 -> n' *i = n/1, M' = M*i*eta/3
  n' *i = n/1 -> n_Gearbox [rpm]/1
  M' = M*i*eta/1 -> M_tire [Nm]/1
  Differential efficiency/1 -> Product/1, Switch/1
  Product/1 -> Switch/3
  Switch/1 -> [Eta_Axle_Drive], M' = M*i*eta/2

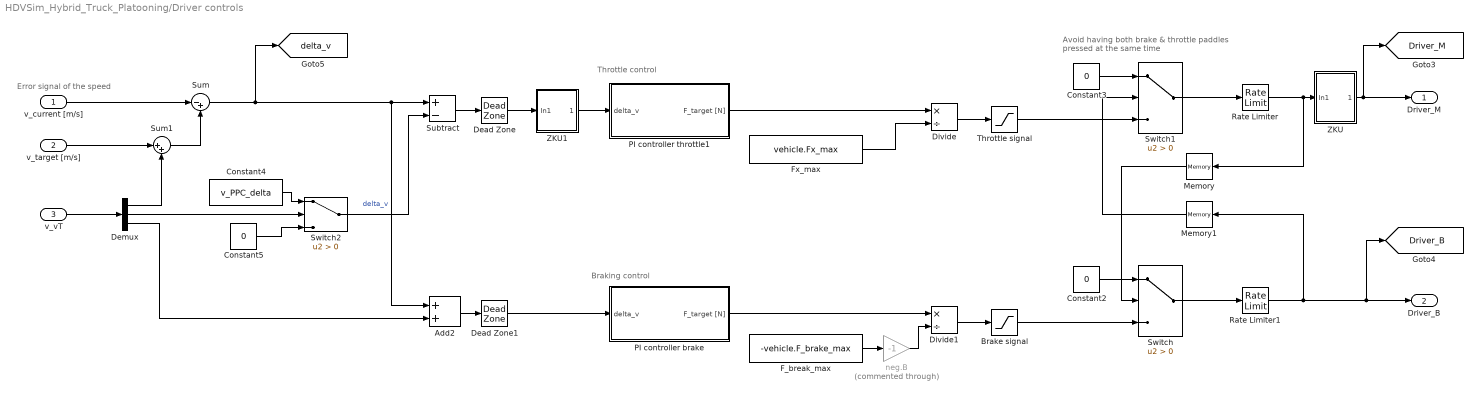
== system HDVSim_Hybrid_Truck_Platooning/Driver controls ==
  note: Avoid having both brake & throttle
      | paddles pressed at the same time
  note: Throttle control
  note: Braking control
  note: Error signal of the speed
  v_current [m/s] : Inport
  v_target [m/s] : Inport  Port=2
  v_vT : Inport  Port=3
  Add2 : Sum
  Brake signal : Saturate  UpperLimit=1  LowerLimit=0  ZeroCross=off
  Constant2 : Constant  Value=0
  Constant3 : Constant  Value=0
  Constant4 : Constant  Value=v_PPC_delta
  Constant5 : Constant  Value=0
  Dead Zone : DeadZone  LowerValue=-0.1/3.6  UpperValue=0.1/3.6  ZeroCross=off  SaturateOnIntegerOverflow=on
  Dead Zone1 : DeadZone  LowerValue=-0.1/3.6  UpperValue=0  ZeroCross=off  SaturateOnIntegerOverflow=on
  Demux : Demux  Outputs=3
  Divide : Product  Inputs=*/
  Divide1 : Product  Inputs=*/
  F_break_max : Constant  Value=-vehicle.F_brake_max
  Fx_max : Constant  Value=vehicle.Fx_max
  Memory : Memory
  Memory1 : Memory
  PI controller brake : Subsystem
  PI controller throttle1 : Subsystem
  Rate Limiter : RateLimiter  RisingSlewLimit=driver.slew_rate_throttle_in  FallingSlewLimit=driver.slew_rate_throttle_out  SampleTimeMode=inherited
  Rate Limiter1 : RateLimiter  RisingSlewLimit=driver.slew_rate_brake_in*100  FallingSlewLimit=driver.slew_rate_brake_out*100  SampleTimeMode=inherited
  Subtract : Sum  Inputs=+-
  Sum : Sum  Inputs=|-+
  Sum1 : Sum  Inputs=|++
  Switch : Switch  Criteria=u2 > Threshold
  Switch1 : Switch  Criteria=u2 > Threshold
  Switch2 : Switch  Criteria=u2 > Threshold
  Throttle signal : Saturate  UpperLimit=1  LowerLimit=0  ZeroCross=off
  ZKU : Subsystem
  ZKU1 : Subsystem
  neg.B : Gain  Commented=through  Gain=-1
  Driver_M : Outport
  Driver_B : Outport  Port=2
  tag scope: Driver_B=global, Driver_M=global, delta_v=global
  wires:
  Sum1/1 -> Sum/2
  v_current [m/s]/1 -> Sum/1
  Fx_max/1 -> Divide/2
  neg.B/1 -> Divide1/2
  Sum/1 -> [delta_v], Add2/1, Subtract/1  "delta_v"
  Divide1/1 -> Brake signal/1
  Divide/1 -> Throttle signal/1
  F_break_max/1 -> neg.B/1
  Switch/1 -> Rate Limiter1/1
  Brake signal/1 -> Switch/3
  Constant2/1 -> Switch/1
  Switch1/1 -> Rate Limiter/1
  Throttle signal/1 -> Switch1/3
  Rate Limiter1/1 -> Memory1/1, [Driver_B], Driver_B/1
  Rate Limiter/1 -> ZKU/1(In1), Memory/1
  Constant3/1 -> Switch1/1
  PI controller throttle1/1(F_target [N]) -> Divide/1
  Dead Zone/1 -> ZKU1/1(In1)
  Dead Zone1/1 -> PI controller brake/1(delta_v)
  PI controller brake/1(F_target [N]) -> Divide1/1
  ZKU/1(Out1) -> [Driver_M], Driver_M/1
  ZKU1/1(Out1) -> PI controller throttle1/1(delta_v)
  Memory/1 -> Switch/2
  Memory1/1 -> Switch1/2
  v_vT/1 -> Demux/1
  Switch2/1 -> Subtract/2
  Demux/2 -> Switch2/2
  Constant4/1 -> Switch2/1
  Constant5/1 -> Switch2/3
  Subtract/1 -> Dead Zone/1
  Demux/1 -> Sum1/2
  v_target [m/s]/1 -> Sum1/1
  Demux/3 -> Add2/2
  Add2/1 -> Dead Zone1/1

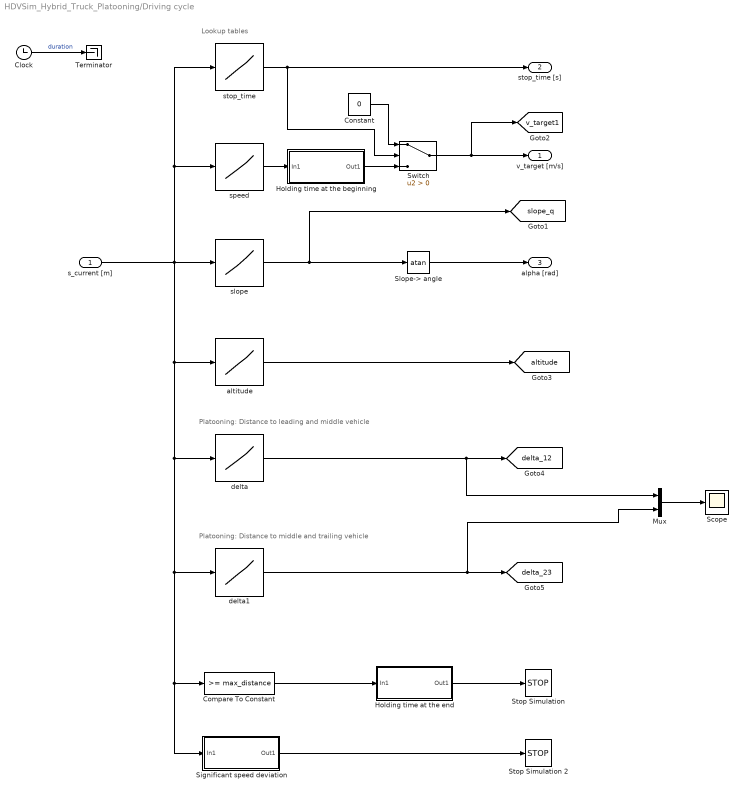
== system HDVSim_Hybrid_Truck_Platooning/Driving cycle ==
  note: Platooning: Distance to leading and middle vehicle
  note: Lookup tables
  note: Platooning: Distance to middle and trailing vehicle
  s_current [m] : Inport
  Clock : Clock
  Compare To Constant : simulink/Logic and Bit Operations/Compare To Constant  relop=>=  const=max_distance  OutDataTypeStr=boolean
  Constant : Constant  Value=0
  Holding time at the beginning : Subsystem
  Holding time at the end : Subsystem
  Mux : Mux  Inputs=2
  Scope : Scope
  Significant speed deviation : Subsystem
  Slope-> angle : Trigonometry  Operator=atan
  Stop Simulation : Stop
  Stop Simulation 2 : Stop
  Switch : Switch  Criteria=u2 > Threshold
  Terminator : Terminator
  altitude : Lookup_n-D  NumberOfTableDimensions=1  BreakpointsForDimension1=cycle.distance  Table=cycle.altitude  InterpMethod=Flat  RndMeth=Simplest  InputSameDT=on
  delta : Lookup_n-D  NumberOfTableDimensions=1  BreakpointsForDimension1=cycle.distance  BeginIndexSearchUsingPreviousIndexResult=on  Table=cycle.delta12  InterpMethod=Flat  RndMeth=Simplest  InputSameDT=on
  delta1 : Lookup_n-D  NumberOfTableDimensions=1  BreakpointsForDimension1=cycle.distance  BeginIndexSearchUsingPreviousIndexResult=on  Table=cycle.delta23  InterpMethod=Flat  RndMeth=Simplest  InputSameDT=on
  slope : Lookup_n-D  NumberOfTableDimensions=1  BreakpointsForDimension1=cycle.distance  Table=cycle.slope  InterpMethod=Flat  RndMeth=Simplest  InputSameDT=on
  speed : Lookup_n-D  NumberOfTableDimensions=1  BreakpointsForDimension1=cycle.distance  Table=cycle.speed  InterpMethod=Flat  RndMeth=Simplest  InputSameDT=on
  stop_time : Lookup_n-D  NumberOfTableDimensions=1  BreakpointsForDimension1=cycle.distance  Table=cycle.stop_time  InterpMethod=Flat  RndMeth=Simplest  InputSameDT=on
  v_target [m/s] : Outport
  stop_time [s] : Outport  Port=2
  alpha [rad] : Outport  Port=3
  tag scope: altitude=global, delta_12=global, delta_23=global, slope_q=global, v_target1=global
  wires:
  slope/1 -> Slope-> angle/1, [slope_q]
  Slope-> angle/1 -> alpha [rad]/1
  Compare To Constant/1 -> Holding time at the end/1(In1)
  Clock/1 -> Terminator/1  "duration"
  Switch/1 -> [v_target1], v_target [m/s]/1
  stop_time/1 -> stop_time [s]/1, Switch/2
  speed/1 -> Holding time at the beginning/1(In1)
  Holding time at the end/1(Out1) -> Stop Simulation/1
  Holding time at the beginning/1(Out1) -> Switch/3
  Constant/1 -> Switch/1
  altitude/1 -> [altitude]
  Significant speed deviation/1(Out1) -> Stop Simulation 2/1
  delta/1 -> Mux/1, [delta_12]
  s_current [m]/1 -> slope/1, delta/1, delta1/1, Significant speed deviation/1(In1), Compare To Constant/1, altitude/1, speed/1, stop_time/1
  delta1/1 -> Mux/2, [delta_23]
  Mux/1 -> Scope/1

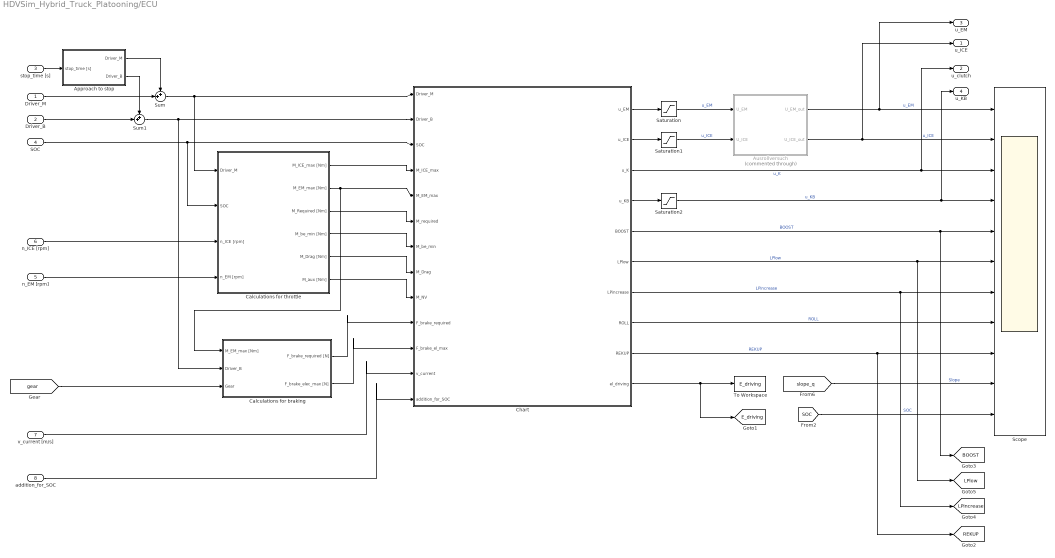
== system HDVSim_Hybrid_Truck_Platooning/ECU ==
  Driver_M : Inport
  Driver_B : Inport  Port=2
  stop_time [s] : Inport  Port=3
  SOC : Inport  Port=4
  n_EM [rpm] : Inport  Port=5
  n_ICE [rpm] : Inport  Port=6
  v_current [m/s] : Inport  Port=7
  addition_for_SOC : Inport  Port=8
  Approach to stop : Subsystem
  Ausrollversuch : Subsystem  Commented=through
  Calculations for braking : Subsystem
  Calculations for throttle : Subsystem
  Chart : Stateflow chart  TreatAsAtomicUnit=on
  Saturation : Saturate  UpperLimit=1  LowerLimit=-1
  Saturation1 : Saturate  UpperLimit=1  LowerLimit=0
  Saturation2 : Saturate  UpperLimit=1  LowerLimit=0
  Scope : Scope  NumInputPorts=11
  Sum : Sum  Inputs=++|
  Sum1 : Sum  Inputs=++|
  To Workspace : ToWorkspace  VariableName=E_driving  SampleTime=-1
      settings: Decimation=10
  u_ICE : Outport
  u_clutch : Outport  Port=2
  u_EM : Outport  Port=3
  u_KB : Outport  Port=4
  tag scope: BOOST=global, E_driving=global, LPincrease=global, LPlow=global, REKUP=global
  wires:
  Chart/1(u_EM) -> Saturation/1
  Chart/2(u_ICE) -> Saturation1/1
  Chart/4(u_KB) -> Saturation2/1
  Sum1/1 -> Calculations for braking/2(Driver_B), Chart/2(Driver_B)
  Sum/1 -> Calculations for throttle/1(Driver_M), Chart/1(Driver_M)
  Chart/3(u_K) -> u_clutch/1, Scope/3  "u_K"
  Calculations for braking/2(F_brake_elec_max [N]) -> Chart/11(F_brake_el_max)
  Calculations for braking/1(F_brake_required [N]) -> Chart/10(F_brake_required)
  SOC/1 -> Calculations for throttle/2(SOC), Chart/3(SOC)
  n_ICE [rpm]/1 -> Calculations for throttle/3(n_ICE [rpm])
  Calculations for throttle/1(M_ICE_max [Nm]) -> Chart/4(M_ICE_max)
  Calculations for throttle/3(M_Required [Nm]) -> Chart/6(M_required)
  Ausrollversuch/2(U_ICE_out) -> Scope/2, u_ICE/1  "u_ICE"
  Saturation2/1 -> u_KB/1, Scope/4  "u_KB"
  Calculations for throttle/5(M_Drag [Nm]) -> Chart/8(M_Drag)
  Calculations for throttle/4(M_be_min [Nm]) -> Chart/7(M_be_min)
  Chart/5(BOOST) -> [BOOST], Scope/5  "BOOST"
  Chart/8(ROLL) -> Scope/8  "ROLL"
  Chart/9(REKUP) -> [REKUP], Scope/9  "REKUP"
  Chart/7(LPincrease) -> [LPincrease], Scope/7  "LPincrease"
  [slope_q] -> Scope/10  "Slope"
  Calculations for throttle/6(M_aux [Nm]) -> Chart/9(M_NV)
  Chart/6(LPlow) -> [LPlow], Scope/6  "LPlow"
  Calculations for throttle/2(M_EM_max [Nm]) -> Calculations for braking/1(M_EM_max [Nm]), Chart/5(M_EM_max)
  [SOC] -> Scope/11  "SOC"
  Ausrollversuch/1(U_EM_out) -> u_EM/1, Scope/1  "u_EM"
  stop_time [s]/1 -> Approach to stop/1(stop_time [s])
  Approach to stop/2(Driver_B) -> Sum1/1
  Approach to stop/1(Driver_M) -> Sum/1
  Driver_M/1 -> Sum/2
  Driver_B/1 -> Sum1/2
  n_EM [rpm]/1 -> Calculations for throttle/4(n_EM [rpm])
  [gear] -> Calculations for braking/3(Gear)
  v_current [m/s]/1 -> Chart/12(v_current)
  Chart/10(el_driving) -> [E_driving], To Workspace/1
  addition_for_SOC/1 -> Chart/13(addition_for_SOC)
  Saturation1/1 -> Ausrollversuch/2(U_ICE)  "u_ICE"
  Saturation/1 -> Ausrollversuch/1(U_EM)  "u_EM"

== system HDVSim_Hybrid_Truck_Platooning/Electric motor ==
  note: Effective motor power
  note: Electric torque
  u_EM : Inport
  n_EM [rpm] : Inport  Port=2
  U_Bat [V] : Inport  Port=3
  Abs : Abs
  Abs1 : Abs
  Divide : Product  Inputs=*/
  Electric machine efficiency mapping : Lookup_n-D  BreakpointsForDimension1=em.efficiency.torque  BreakpointsForDimension2=em. efficiency.speed  Table=em.efficiency.characteristic_map  RndMeth=Simplest  InputSameDT=on
  Electric machine efficiency mapping2 : Lookup_n-D  BreakpointsForDimension1=em.efficiency.torque  BreakpointsForDimension2=em. efficiency.speed  Table=em.efficiency.characteristic_map  RndMeth=Simplest  InputSameDT=on
  Gain : Gain  Gain=2*pi/60
  Machine current demand : Subsystem
  Machine torque demand : Subsystem
  Math Function : Math  Operator=reciprocal  SaturateOnIntegerOverflow=on
  Product1 : Product
  Product2 : Product  Inputs=3
  Saturation : Saturate  UpperLimit=Bat.Useable_capacity / Bat.Useable_range*10  LowerLimit=-Bat.Useable_capacity / Bat.Useable_range*10
  Saturation1 : Saturate  UpperLimit=inf  LowerLimit=1
  Speed-torrque characteristics : Lookup_n-D  NumberOfTableDimensions=1  BreakpointsForDimension1=em.speed  Table=em.trq  ExtrapMethod=Clip  RndMeth=Simplest  InputSameDT=on
  Switch : Switch
  M_EM [Nm] : Outport
  I_EM_current [A] : Outport  Port=2
  tag scope: M_EM=global, n_EM=global, u_EM=global
  wires:
  Speed-torrque characteristics/1 -> Product1/1  "M_EM_max"
  u_EM/1 -> Product1/2, [u_EM]
  U_Bat [V]/1 -> Divide/2, Machine torque demand/4(U_Bat [V]), Machine current demand/4(U_Bat [V])  "U_Bat [V]"
  Machine current demand/1(I_target [A]) -> Saturation/1
  Saturation/1 -> Machine torque demand/2(I_current [A])
  Machine torque demand/1(M_EM [Nm]) -> Abs/1, Product2/3, [M_EM], M_EM [Nm]/1, Switch/2
  Gain/1 -> Product2/2
  Divide/1 -> I_EM_current [A]/1
  Math Function/1 -> Switch/1
  Electric machine efficiency mapping/1 -> Switch/3, Math Function/1  "Eta_EM"
  Switch/1 -> Product2/1
  Product2/1 -> Divide/1
  Abs/1 -> Electric machine efficiency mapping/1
  Product1/1 -> Machine current demand/2(M_EM_target [Nm]), Abs1/1  "M_EM_targetl"
  n_EM [rpm]/1 -> Electric machine efficiency mapping2/2, Saturation1/1, Electric machine efficiency mapping/2, Machine torque demand/1(n_EM [rpm]), Machine current demand/1("n_EM "), [n_EM], Speed-torrque characteristics/1  "n_EM [1/min]"
  Abs1/1 -> Electric machine efficiency mapping2/1
  Electric machine efficiency mapping2/1 -> Machine current demand/3(Eff_EM), Machine torque demand/3(Eff_EM)  "ETA_EM"
  Saturation1/1 -> Gain/1

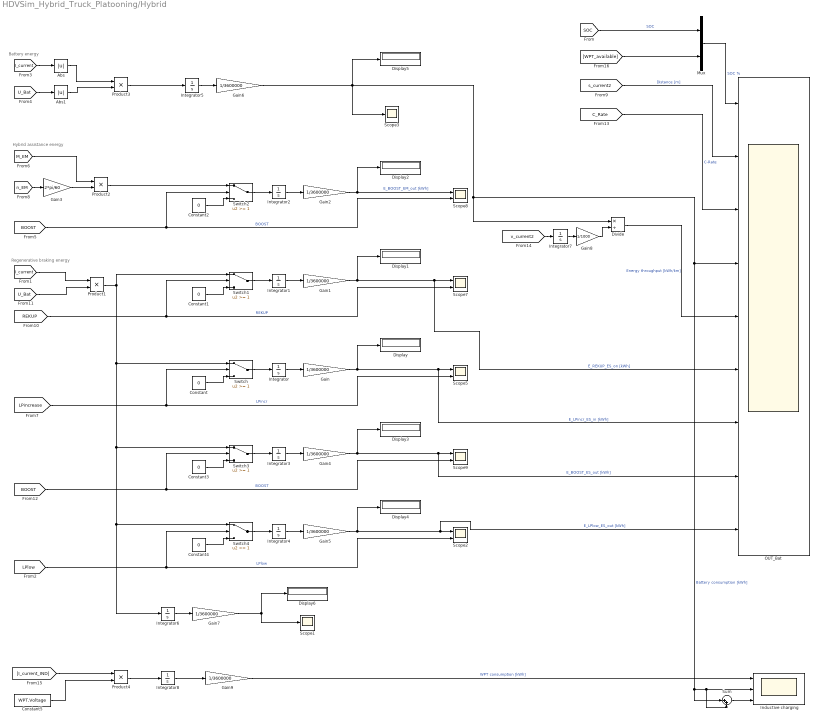
== system HDVSim_Hybrid_Truck_Platooning/Hybrid ==
  note: Regenerative braking energy
  note: Hybrid assistance energy
  note: Battery energy
  Abs : Abs
  Abs1 : Abs
  Constant{,1..4} (5 alike) : Constant  Value=0
  Constant5 : Constant  Value=WPT.Voltage
  Display{,1..6} (7 alike) : Display
  Divide : Product  Inputs=*/
  Gain{,1..2,4..7,9} (8 alike) : Gain  Gain=1/3600000
  Gain3 : Gain  Gain=2*pi/60
  Gain8 : Gain  Gain=1/1000
  Inductive charging : Scope  NumInputPorts=3
  Integrator{,1..6,8} (8 alike) : Integrator
  Integrator7 : Integrator  InitialCondition=0.00000001
  Mux : Mux  Inputs=2
  OUT_Bat : Scope  NumInputPorts=9
  Product{1..4} (4 alike) : Product
  Scope1 : Scope
  Scope{2,5,7..9} (5 alike) : Scope  NumInputPorts=2
  Scope3 : Scope
  Sum : Sum  Inputs=|++
  Switch{,1..4} (5 alike) : Switch  Threshold=1
  wires:
  Product1/1 -> Switch1/1, Switch/1, Switch3/1, Integrator6/1, Switch4/1
  Gain5/1 -> OUT_Bat/9, Scope2/1, Display4/1  "E_LPlow_ES_out [kWh]"
  Constant4/1 -> Switch4/3
  Integrator4/1 -> Gain5/1
  Switch4/1 -> Integrator4/1
  [LPlow] -> Scope2/2, Switch4/2  "LPlow"
  Gain4/1 -> OUT_Bat/8, Scope9/1, Display3/1  "E_BOOST_ES_out [kWh]"
  Constant3/1 -> Switch3/3
  Integrator3/1 -> Gain4/1
  Switch3/1 -> Integrator3/1
  [BOOST] -> Scope9/2, Switch3/2  "BOOST"
  Gain3/1 -> Product2/2
  [n_EM] -> Gain3/1
  Gain2/1 -> Scope8/1, Display2/1  "E_BOOST_EM_out [kWh]"
  Constant2/1 -> Switch2/3
  Integrator2/1 -> Gain2/1
  Switch2/1 -> Integrator2/1
  [BOOST] -> Scope8/2, Switch2/2  "BOOST"
  Product2/1 -> Switch2/1
  Gain1/1 -> OUT_Bat/6, Scope7/1, Display1/1  "E_REKUP_ES_on [kWh]"
  Constant1/1 -> Switch1/3
  Integrator1/1 -> Gain1/1
  Switch1/1 -> Integrator1/1
  [REKUP] -> Scope7/2, Switch1/2  "REKUP"
  [U_Bat] -> Product1/2
  [I_current] -> Product1/1
  Gain/1 -> OUT_Bat/7, Scope5/1, Display/1  "E_LPincr_ES_in [kWh]"
  Constant/1 -> Switch/3
  Integrator/1 -> Gain/1
  Switch/1 -> Integrator/1
  [LPincrease] -> Scope5/2, Switch/2  "LPincr"
  [M_EM] -> Product2/1
  [SOC] -> Mux/1  "SOC"
  Gain7/1 -> Display6/1, Scope1/1
  Integrator6/1 -> Gain7/1
  [U_Bat] -> Abs1/1
  [I_current] -> Abs/1
  Product3/1 -> Integrator5/1
  Integrator5/1 -> Gain6/1
  Abs/1 -> Product3/1
  Abs1/1 -> Product3/2
  [s_current2] -> OUT_Bat/2  "Distance [m]"
  [C_Rate] -> OUT_Bat/3  "C-Rate"
  Divide/1 -> OUT_Bat/5  "Energy throughput [kWh/km]"
  [v_current2] -> Integrator7/1
  Integrator7/1 -> Gain8/1
  Gain8/1 -> Divide/2
  Gain6/1 -> Scope3/1, Sum/1, Sum/2, Inductive charging/2, OUT_Bat/4, Divide/1, Display5/1  "Battery consumption [kWh]"
  [I_current_IND] -> Product4/1
  Constant5/1 -> Product4/2
  Product4/1 -> Integrator8/1
  Gain9/1 -> Inductive charging/1  "WPT consumption [kWh]"
  Integrator8/1 -> Gain9/1
  Sum/1 -> Inductive charging/3
  [WPT_available] -> Mux/2
  Mux/1 -> OUT_Bat/1  "SOC %"

== system HDVSim_Hybrid_Truck_Platooning/ICE engine ==
  note: Engine loading
  note: Consumption calculations
  u_ICE : Inport
  n_ICE [rpm] : Inport  Port=2
  Additional consumptions : Subsystem
  Consumption : Subsystem
  Drag torque : Lookup  InputValues=engine.drag_torque.speed  Table=engine.drag_torque.trq  LookUpMeth=Interpolation-Use End Values
  Full load curve : Lookup  InputValues=engine.full_load.speed  Table=engine.full_load.trq  LookUpMeth=Interpolation-Use End Values
  MinMax : MinMax  Inputs=2
  Product1 : Product
  Sum : Sum  Inputs=|+-
  Sum1 : Sum  Inputs=|++
  maximum engine torque due to tire slip : Subsystem
  M_ICE [Nm] : Outport
  tag scope: M_mot=global, n_mot=global
  wires:
  n_ICE [rpm]/1 -> Additional consumptions/2(n_clutch_en [rpm]), Consumption/2(n [rpm]), [n_mot], Drag torque/1, Full load curve/1
  Sum/1 -> Product1/2
  Product1/1 -> Sum1/1
  Drag torque/1 -> Sum1/2, Sum/2  "M_Drag"
  Additional consumptions/1(M_ICE_aftr_aux [Nm]) -> M_ICE [Nm]/1
  u_ICE/1 -> Product1/1
  Full load curve/1 -> MinMax/2  "M_ICE_max"
  Sum1/1 -> [M_mot], Additional consumptions/1(M_ICE_bfor_aux [Nm]), Consumption/1(M [Nm])
  maximum engine torque due to tire slip/1(M_mot_max_traction [Nm]) -> MinMax/1
  MinMax/1 -> Sum/1

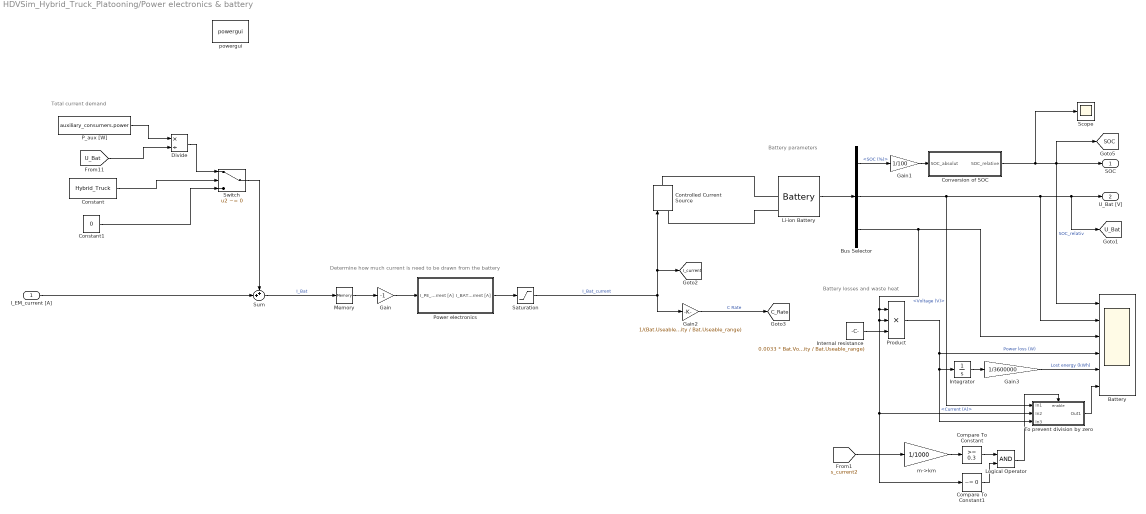
== system HDVSim_Hybrid_Truck_Platooning/Power electronics & battery ==
  note: Battery parameters
  note: Battery losses and waste heat
  note: Total current demand
  note: Determine how much current is need to be drawn from the battery
  I_EM_current [A] : Inport
  Battery : Scope  NumInputPorts=6
  Bus Selector : BusSelector  OutputSignals=SOC (%),Voltage (V),Current (A)
  Compare To Constant : simulink/Logic and Bit Operations/Compare To Constant  relop=>=  const=0.3  OutDataTypeStr=uint8  ZeroCross=off
  Compare To Constant1 : simulink/Logic and Bit Operations/Compare To Constant  relop=~=  const=0  OutDataTypeStr=uint8  ZeroCross=off
  Constant : Constant  Value=Hybrid_Truck
  Constant1 : Constant  Value=0
  Controlled Current Source : powerlib/Electrical Sources/Controlled Current Source  Initialize=off  Source_Type=DC  Amplitude=0  Phase=0  Frequency=0  Measurements=None
      settings: SourceProductName=Simscape Electrical
  Conversion of SOC : Subsystem
  Divide : Product  Inputs=*/
  Gain : Gain  Gain=-1
  Gain1 : Gain  Gain=1/100
  Gain2 : Gain  Gain=1/(Bat.Useable_capacity / Bat.Useable_range)
  Gain3 : Gain  Gain=1/3600000
  Integrator : Integrator
  Internal resistance : Constant  Value=0.0033 * Bat.Voltage / (Bat.Useable_capacity / Bat.Useable_range)
  Li-ion Battery : electricdrivelib/Extra Sources/Battery  BatType=Lithium-Ion  ShowTempParam=on  ThermalPreset=no  ShowAgeParam=off  NomV=Bat.Voltage  NomQ=Bat.Useable_capacity / Bat.Useable_range  SOC=(Bat.SOC_start *Bat.Useable_range+(0.5-Bat.Useable_range/2))* 100  Batt_Tr=30  PresetModel=off  MaxQ=Bat.Useable_capacity / Bat.Useable_range *8077/7500  MinV=487.5  FullV=Bat.Voltage * 1.178  Dis_rate=Bat.Useable_capacity / Bat.Useable_range * 1  R=0.0033 * Bat.Voltage / (Bat.Useable_capacity / Bat.Useable_range)  Normal_OP=Bat.Useable_capacity / Bat.Useable_range * 0.962  expZone="[Bat.Voltage*4339/4000     Bat.Useable_capacity / Bat.Useable_range/5]"  current=[5 25 50 250]  Units=Ampere-hour  Tci=20  NomT=20  T2=-30  MaxQ2=Bat.Useable_capacity / Bat.Useable_range *8077/7500  FullV2=Bat.Voltage * 1.178  Normal_OP2=487.5  expZone2="[Bat.Voltage*4339/4000     Bat.Useable_capacity / Bat.Useable_range/5]"  Rca=0.6  ti=1000  Dp=0  Neq0=0  Tsim=1e6  Ta1=25  Qeol=5.4*0.9  Reol=0.013333*1.2  Char_age=[2.3478, 3]  Dis_age=[2.3478, 10]  N1=1500  N2=10500  N3=1000  N4=1400  Ta2=45  N5=950
      settings: SourceProductName=Simscape Electrical
  Logical Operator : Logic  AllPortsSameDT=off  OutDataTypeStr=boolean
  Memory : Memory
  P_aux [W] : Constant  Value=auxiliary_consumers.power
  Power electronics : Subsystem
  Product : Product  Inputs=3
  Saturation : Saturate  UpperLimit=450  LowerLimit=-450
  Scope : Scope
  Sum : Sum  Inputs=++|
  Switch : Switch  Criteria=u2 ~= 0
  To prevent division by zero : Subsystem
  m->km : Gain  Gain=1/1000
  powergui : powerlib/powergui  Priority=1  SimulationMode=Discrete  SampleTime=sample_time  frequency=60  Iterations=50  frequencyindice=0  Pbase=100e6  ErrMax=1e-4  UnitsV=kV  UnitsW=MW  buscounter=0  FunctionMessages=off  echomessages=off  EnableUseOfTLC=off  CurrentSourceSwitches=off  DisableSnubberDevices=off  DisableRonSwitches=off  DisableVfSwitches=off  DisplayEquations=off  SolverType=Tustin  Interpol=off  ExternalGateDelay=off  methode=off  Ts=100  x0status=blocks  SPID=off  SwTol=0  HookPort=off  RestoreLinks=warning  ResistiveCurrentMeasurement=off  Frange=[0:2:500]  Ylog=off  Xlog=on  ShowGrid=off  save=off  variable=ZData  structure=0  ZoomFFT=off  StartTime=0.0  cycles=1  DisplayStyle=1  fundamental=60  FreqAxis=off  MaxFrequency=1000  frequencyindicesteady=1  RmsSteady=1  display=off
  SOC : Outport
  U_Bat [V] : Outport  Port=2
  tag scope: C_Rate=global, I_current=global, SOC=global, U_Bat=global
  wires:
  Li-ion Battery/1 -> Bus Selector/1
  Bus Selector/1 -> Gain1/1  "<SOC (%)>"
  Bus Selector/2 -> To prevent division by zero/1(In1), U_Bat [V]/1, [U_Bat], Battery/2  "<Voltage (V)>"
  Gain1/1 -> Conversion of SOC/1(SOC_absolut)
  Conversion of SOC/1(SOC_relative) -> Scope/1, SOC/1, [SOC], Battery/1  "SOC_relativ"
  I_EM_current [A]/1 -> Sum/2
  Saturation/1 -> Gain2/1, Controlled Current Source/1, [I_current]  "I_Bat_current"
  Gain2/1 -> [C_Rate]  "C Rate"
  [U_Bat] -> Divide/2
  P_aux [W]/1 -> Divide/1
  Constant/1 -> Switch/2
  Divide/1 -> Switch/1
  Constant1/1 -> Switch/3
  Switch/1 -> Sum/1
  Bus Selector/3 -> Product/1, Compare To Constant1/1, To prevent division by zero/2(In2), Product/2, Battery/3  "<Current (A)>"
  Internal resistance/1 -> Product/3
  Product/1 -> Battery/4, To prevent division by zero/3(In3), Integrator/1  "Power loss (W)"
  Integrator/1 -> Gain3/1
  Gain3/1 -> Battery/5  "Lost energy (kWh)"
  [s_current2] -> m->km/1
  m->km/1 -> Compare To Constant/1
  To prevent division by zero/1(Out1) -> Battery/6
  Compare To Constant/1 -> Logical Operator/1
  Compare To Constant1/1 -> Logical Operator/2
  Logical Operator/1 -> To prevent division by zero/Enable
  Gain/1 -> Power electronics/1(I_PE_current [A])
  Sum/1 -> Memory/1  "I_Bat"
  Memory/1 -> Gain/1
  Power electronics/1(I_BAT_current [A]) -> Saturation/1
  connections:
  Li-ion Battery/LConn1 -- Controlled Current Source/RConn1
  Li-ion Battery/LConn2 -- Controlled Current Source/LConn1

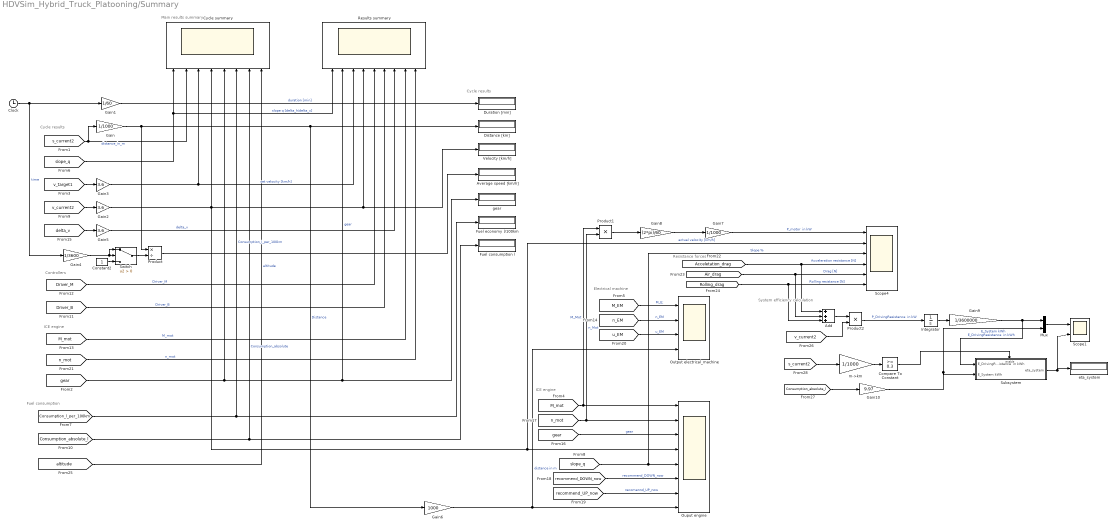
== system HDVSim_Hybrid_Truck_Platooning/Summary ==
  note: System efficiency calculation
  note: Resistance forces
  note: Electrical machine
  note: ICE engine
  note: Main results summary
  note: Cycle results
  note: Fuel consumption
  note: ICE engine
  note: Controllers
  note: Cycle results
  Add : Sum  Inputs=+++
  Average speed [km/h] : Display
  Clock : Clock
  Compare To Constant : simulink/Logic and Bit Operations/Compare To Constant  relop=>=  const=0.3  OutDataTypeStr=uint8  ZeroCross=off
  Constant2 : Constant
  Cycle summary : Scope  NumInputPorts=8
  Distance [km] : Display
  Duration [min] : Display
  Fuel consumption l : Display
  Fuel economy l/100km : Display
  Gain : Gain  Gain=1/1000
  Gain1 : Gain  Gain=1/60
  Gain10 : Gain  Gain=9.97
  Gain2 : Gain  Gain=3.6
  Gain3 : Gain  Gain=3.6
  Gain4 : Gain  Gain=1/3600
  Gain5 : Gain  Gain=3.6
  Gain6 : Gain  Gain=1000
  Gain7 : Gain  Gain=1/1000
  Gain8 : Gain  Gain=(2*pi)/60
  Gain9 : Gain  Gain=1/3600000
  Integrator : Integrator
  Mux : Mux  Inputs=2
  Ouput engine : Scope  NumInputPorts=8
  Output electrical_machine : Scope  NumInputPorts=4
  Product : Product  Inputs=*/  RndMeth=Zero
  Product1 : Product
  Product2 : Product
  Results summary : Scope  NumInputPorts=9
  Scope1 : Scope  NumInputPorts=2
  Scope4 : Scope  NumInputPorts=6
  Subsystem : Subsystem
  Switch : Switch  Criteria=u2 > Threshold
  Velocity [km/h] : Display
  eta_system : Display
  gear : Display
  m->km : Gain  Gain=1/1000
  wires:
  [v_current2] -> Gain2/1
  [s_current2] -> Cycle summary/2, Gain/1  "distance_in_m"
  Gain/1 -> Distance [km]/1, Gain6/1, Product/1  "Distance"
  Clock/1 -> Gain1/1, Gain4/1  "time"
  Gain1/1 -> Duration [min]/1  "duration [min]"
  Gain2/1 -> Ouput engine/4, Scope4/2, Results summary/4, Velocity [km/h]/1, Cycle summary/4  "actual velocity [km/h]"
  [gear] -> gear/1, Results summary/2, Cycle summary/5  "gear"
  [v_target1] -> Gain3/1
  [slope_q] -> Results summary/1, Cycle summary/1  "slope q [delta_h/delta_x]"
  [Consumption_l_per_100km] -> Cycle summary/6, Fuel economy l/100km/1  "Consumption_l_per_100km"
  Gain3/1 -> Cycle summary/3, Results summary/3  "set velocity [km/h]"
  Product/1 -> Average speed [km/h]/1
  [Consumption_absolute_l] -> Cycle summary/7, Fuel consumption l/1  "Consumption_absolute"
  [Driver_M] -> Results summary/5  "Driver_M"
  [Driver_B] -> Results summary/6  "Driver_B"
  [M_mot] -> Results summary/8  "M_mot"
  [delta_v] -> Gain5/1
  [M_mot] -> Ouput engine/1, Product1/1  "M_Mot"
  [n_mot] -> Ouput engine/2, Product1/2  "n_Mot"
  [gear] -> Ouput engine/3  "gear"
  [recommend_DOWN_now] -> Ouput engine/6  "recommend_DOWN_now"
  [recommend_UP_now] -> Ouput engine/7  "recomennd_UP_now"
  [slope_q] -> Ouput engine/5, Scope4/3  "Slope %"
  Gain5/1 -> Results summary/7  "delta_v"
  [n_mot] -> Results summary/9  "n_mot"
  [M_EM] -> Output electrical_machine/1  "M_E;"
  [n_EM] -> Output electrical_machine/2  "n_EM"
  [u_EM] -> Output electrical_machine/3  "u_EM"
  Product1/1 -> Gain8/1
  Gain7/1 -> Scope4/1  "P_motor  in kW"
  [Acceletation_drag] -> Add/1, Scope4/4  "Acceleration resistance [N]"
  [Air_drag] -> Add/2, Scope4/5  "Drag [N]"
  [Rolling_drag] -> Add/3, Scope4/6  "Rolling resistance [N]"
  Gain4/1 -> Switch/1, Switch/2
  Constant2/1 -> Switch/3
  Switch/1 -> Product/2
  [altitude] -> Cycle summary/8  "altitude"
  Gain6/1 -> Output electrical_machine/4, Ouput engine/8  "distance in m"
  Gain8/1 -> Gain7/1
  Add/1 -> Product2/1
  [v_current2] -> Product2/2
  Product2/1 -> Integrator/1  "P_DrivingResistance  in kW"
  Integrator/1 -> Gain9/1
  Gain9/1 -> Subsystem/1(E_DrivingResistance  in kWh), Mux/1  "E_DrivingResistance  in kWh"
  [Consumption_absolute_l] -> Gain10/1
  Gain10/1 -> Mux/2, Subsystem/2(E_System kWh)  "E_System kWh"
  Mux/1 -> Scope1/1
  [s_current2] -> m->km/1
  m->km/1 -> Compare To Constant/1
  Subsystem/1(eta_system) -> Scope1/2, eta_system/1
  Compare To Constant/1 -> Subsystem/Enable

== system HDVSim_Hybrid_Truck_Platooning/Tires ==
  M_tire [Nm] : Inport
  v_current [m/s] : Inport  Port=2
  F=M/r : Product  Inputs=*/
  Tire radius : Constant  Value=tires.radius
  "phi. -> n[1/min]" : Gain  Gain=60/2/pi
  phi. = v/r : Product  Inputs=/*
  n_tire [rpm] : Outport
  F_x [N] : Outport  Port=2
  wires:
  phi. = v/r/1 -> "phi. -> n[1/min]"/1
  "phi. -> n[1/min]"/1 -> n_tire [rpm]/1
  Tire radius/1 -> F=M/r/2, phi. = v/r/1
  v_current [m/s]/1 -> phi. = v/r/2
  M_tire [Nm]/1 -> F=M/r/1
  F=M/r/1 -> F_x [N]/1

== system HDVSim_Hybrid_Truck_Platooning/Transmission ==
  note: Transmission torque multiplication through the different gears
  M_EM [Nm] : Inport
  M_clutch_dis [Nm] : Inport  Port=2
  n_Gearbox [rpm] : Inport  Port=3
  alpha : Inport  Port=4
  Determine when shifting occurs : Subsystem  TreatAsAtomicUnit=on
  Memory1 : Memory
  Number of gears : Constant  Value=length(transmission.ratios)
  Saturation : Saturate  UpperLimit=2000  LowerLimit=0
  Shifting strategy : Stateflow chart  TreatAsAtomicUnit=on
  Sum : Sum
  Torque flow through the transmission : Subsystem
  ZKU : Subsystem
  init_gear : Constant  Value=transmission.init_gear
  n_clutch_dis [rpm] : Outport
  M_Gearbox [Nm] : Outport  Port=2
  tag scope: gear=global, i_gearbox=global, recommend_DOWN_now=global, recommend_UP_now=global
  wires:
  n_Gearbox [rpm]/1 -> Torque flow through the transmission/2(n_gearbox_out [1/min]), Determine when shifting occurs/2(n_Gear_out [1/min])
  Torque flow through the transmission/2(M_gearbox_out [Nm]) -> [M_Gear_out], M_Gearbox [Nm]/1
  Torque flow through the transmission/1(n_gearbox_in [1/min]) -> Saturation/1
  init_gear/1 -> Shifting strategy/1(init_gear)
  Determine when shifting occurs/27(check_torque_reseve_2lower) -> Shifting strategy/29(check_torque_reserve_2lower)
  Determine when shifting occurs/26(check_torque_reseve_2higher) -> Shifting strategy/28(check_torque_reserve_2higher)
  Determine when shifting occurs/1(reccommend_down_2higher) -> Shifting strategy/3(recommend_down_2higher)
  Determine when shifting occurs/2(reccommend_down_1higher) -> Shifting strategy/4(recommend_down_1higher)
  Determine when shifting occurs/3(reccommend_down_now) -> Shifting strategy/5(recommend_down_now), [recommend_DOWN_now]
  Determine when shifting occurs/4(reccommend_down_1lower) -> Shifting strategy/6(recommend_down_1lower)
  Determine when shifting occurs/5(reccommend_down_2lower) -> Shifting strategy/7(recommend_down_2llower)
  Determine when shifting occurs/6(reccommend_up_2higher) -> Shifting strategy/8(recommend_up_2higher)
  Determine when shifting occurs/7(reccommend_up_1higher) -> Shifting strategy/9(recommend_up_1higher)
  Determine when shifting occurs/8(reccommend_up_now) -> Shifting strategy/10(recommend_up_now), [recommend_UP_now]
  Determine when shifting occurs/9(reccommend_up_1lower) -> Shifting strategy/11(recommend_up_1lower)
  Determine when shifting occurs/10(reccommend_up_2lower) -> Shifting strategy/12(recommend_up_2lower)
  Determine when shifting occurs/11(check_n_min_2higher) -> Shifting strategy/13(check_n_min_2higher)
  Determine when shifting occurs/12(check_n_min_1higher) -> Shifting strategy/14(check_n_min_1higher)
  Determine when shifting occurs/13(check_n_min_now) -> Shifting strategy/15(check_n_min_now)
  Determine when shifting occurs/14(check_n_min_1lower) -> Shifting strategy/16(check_n_min_1lower)
  Determine when shifting occurs/15(check_n_min_2lower) -> Shifting strategy/17(check_n_min_2lower)
  Determine when shifting occurs/16(check_n_max_2higher) -> Shifting strategy/18(check_n_max_2higher)
  Determine when shifting occurs/17(check_n_max_1higher) -> Shifting strategy/19(check_n_max_1higher)
  Determine when shifting occurs/18(check_n_max_now) -> Shifting strategy/20(check_n_max_now)
  Determine when shifting occurs/19(check_n_max_1lower) -> Shifting strategy/21(check_n_max_1lower)
  Determine when shifting occurs/20(check_n_max_2lower) -> Shifting strategy/22(check_n_max_2lower)
  Determine when shifting occurs/21(check_M_max_2higher) -> Shifting strategy/23(check_M_max_2higher)  "check_M_max_2higher"
  Determine when shifting occurs/22(check_M_max_1higher) -> Shifting strategy/24(check_M_max_1higher)  "check_M_max_1higher"
  Determine when shifting occurs/23(check_M_max_now) -> Shifting strategy/25(check_M_max_now)  "check_M_max_now"
  Determine when shifting occurs/24(check_M_max_1lower) -> Shifting strategy/26(check_M_max_1lower)  "check_M_max_1lower"
  Determine when shifting occurs/25(check_M_max_2lower) -> Shifting strategy/27(check_M_max_2lower)  "check_M_max_2lower"
  Memory1/1 -> [Gear], ZKU/1(Gear), Torque flow through the transmission/3(Gear), [gear]
  M_clutch_dis [Nm]/1 -> Sum/2
  Sum/1 -> Torque flow through the transmission/1(M_gearbox_in [Nm])  "M_gearbox_in [Nm]"
  Torque flow through the transmission/3(i_gearbox) -> [i_gearbox]
  Saturation/1 -> n_clutch_dis [rpm]/1
  M_EM [Nm]/1 -> Sum/1, Determine when shifting occurs/4(M_EM [Nm])
  Number of gears/1 -> Shifting strategy/2(z)
  alpha/1 -> Determine when shifting occurs/5(alpha)
  [gear] -> Memory1/1
  Shifting strategy/1(gear) -> [gear]
  [Gear] -> Determine when shifting occurs/1(Gear)
  [M_Gear_out] -> Determine when shifting occurs/3(M_Gear_out [Nm])

== system HDVSim_Hybrid_Truck_Platooning/Vehicle ==
  note: Net tractive force applied on the vehicle
  note: Vehicle acceleration
  F_x [N] : Inport
  u_KB : Inport  Port=2
  alpha [rad] : Inport  Port=3
  Add : Sum  Inputs=-+-
  Breaking force [N] : Product  RndMeth=Zero
  Cargo weight : Constant  Value=vehicle.payload
  Driving resistances without acceleration : Subsystem
  F_brake_max : Constant  Value=vehicle.F_brake_max
  Integrator : Integrator
  Integrator1 : Integrator  InitialCondition=cycle.speed_init  LimitOutput=on  LowerSaturationLimit=0
  Product : Product  Inputs=3
  Product2 : Product  Inputs=*/  RndMeth=Zero
  Product3 : Product  Inputs=**  RndMeth=Zero
  Saturation : Saturate  UpperLimit=15  LowerLimit=-15
  Sum1 : Sum  Inputs=|++
  Sum2 : Sum  Inputs=|++
  Vehicle weight : Constant  Value=vehicle.mass
  v_current [m/s] : Outport
  s_current [m] : Outport  Port=2
  tag scope: Acceletation_drag=global, s_current2=global, v_current2=global
  wires:
  alpha [rad]/1 -> Driving resistances without acceleration/1(alpha [rad])
  Add/1 -> Product2/1
  Driving resistances without acceleration/1(F_W [N]) -> Add/3
  F_x [N]/1 -> Add/2  "F_x"
  F_brake_max/1 -> Breaking force [N]/2
  Integrator/1 -> [s_current2], s_current [m]/1  "s_current"
  Cargo weight/1 -> Sum1/2, Sum2/2
  Sum1/1 -> Product2/2
  Vehicle weight/1 -> Sum2/1, Product3/2
  Product3/1 -> Sum1/1
  Integrator1/1 -> Driving resistances without acceleration/2(v [m/s]), v_current [m/s]/1, Integrator/1, [v_current2]  "v_current"
  [lamda] -> Product/1, Product3/1
  u_KB/1 -> Breaking force [N]/1
  Breaking force [N]/1 -> Add/1  "F_brake"
  Product2/1 -> Saturation/1, Product/3  "a"
  Product/1 -> [Acceletation_drag]
  Sum2/1 -> Product/2  "m_total"
  Saturation/1 -> Integrator1/1

== system HDVSim_Hybrid_Truck_Platooning/Active cruise control/Braking from upper speed limit ==
  v_target [m/s] : Inport
  Add3 : Sum  Inputs=+-
  Constant1 : Constant  Value=90/3.6
  Constant10 : Constant  Value=prospective_cruise_control
  Constant6 : Constant  Value=v_PPC_delta
  Constant7 : Constant  Value=0
  Constant8 : Constant  Value=0
  Saturation Dynamic : simulink/Discontinuities/Saturation Dynamic  OutMin=[]  OutMax=[]  OutDataTypeStr=Inherit: Same as second input  OutDataType=fixdt(1, 16)  OutScaling=2^-10  DoSatur=off
  Switch3 : Switch  Criteria=u2 > Threshold
  Out1 : Outport
  wires:
  Switch3/1 -> Out1/1
  Constant6/1 -> Saturation Dynamic/2
  Constant1/1 -> Add3/1
  Constant7/1 -> Switch3/3
  Add3/1 -> Saturation Dynamic/1
  Constant8/1 -> Saturation Dynamic/3
  Constant10/1 -> Switch3/2
  v_target [m/s]/1 -> Add3/2
  Saturation Dynamic/1 -> Switch3/1

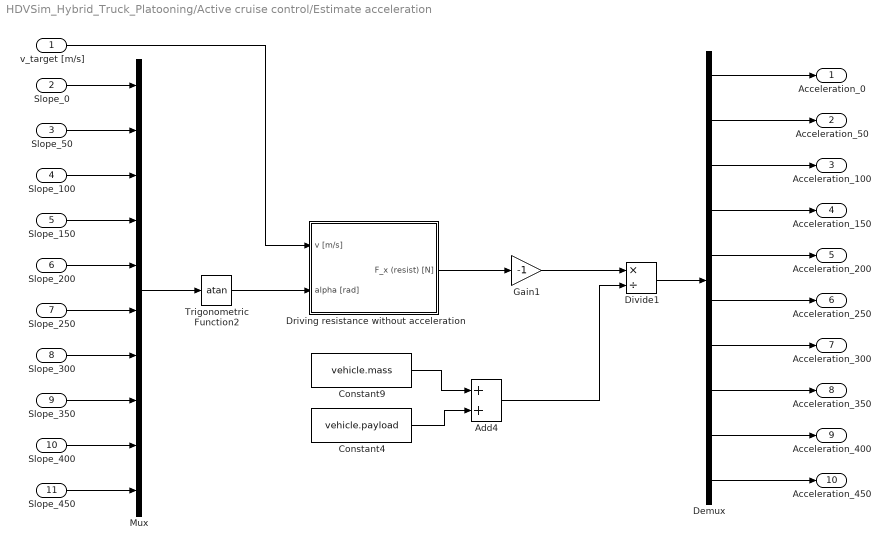
== system HDVSim_Hybrid_Truck_Platooning/Active cruise control/Estimate acceleration ==
  v_target [m/s] : Inport
  Slope_0 : Inport  Port=2
  Slope_50 : Inport  Port=3
  Slope_100 : Inport  Port=4
  Slope_150 : Inport  Port=5
  Slope_200 : Inport  Port=6
  "Slope_250 " : Inport  Port=7
  Slope_300 : Inport  Port=8
  Slope_350 : Inport  Port=9
  Slope_400 : Inport  Port=10
  Slope_450 : Inport  Port=11
  Add4 : Sum
  Constant4 : Constant  Value=vehicle.payload
  Constant9 : Constant  Value=vehicle.mass
  Demux : Demux  Outputs=10
  Divide1 : Product  Inputs=*/
  Driving resistance without acceleration : Subsystem
  Gain1 : Gain  Gain=-1
  Mux : Mux  Inputs=10
  Trigonometric Function2 : Trigonometry  Operator=atan
  Acceleration_0 : Outport
  Acceleration_50 : Outport  Port=2
  Acceleration_100 : Outport  Port=3
  Acceleration_150 : Outport  Port=4
  Acceleration_200 : Outport  Port=5
  Acceleration_250 : Outport  Port=6
  Acceleration_300 : Outport  Port=7
  Acceleration_350 : Outport  Port=8
  Acceleration_400 : Outport  Port=9
  Acceleration_450 : Outport  Port=10
  wires:
  v_target [m/s]/1 -> Driving resistance without acceleration/1(v [m/s])
  Trigonometric Function2/1 -> Driving resistance without acceleration/2(alpha [rad])
  Constant9/1 -> Add4/1
  Constant4/1 -> Add4/2
  Driving resistance without acceleration/1(F_x (resist) [N]) -> Gain1/1
  Add4/1 -> Divide1/2
  Gain1/1 -> Divide1/1
  Mux/1 -> Trigonometric Function2/1
  Divide1/1 -> Demux/1
  Demux/1 -> Acceleration_0/1
  Slope_0/1 -> Mux/1
  Slope_50/1 -> Mux/2
  Slope_100/1 -> Mux/3
  Slope_150/1 -> Mux/4
  Slope_200/1 -> Mux/5
  "Slope_250 "/1 -> Mux/6
  Slope_300/1 -> Mux/7
  Slope_350/1 -> Mux/8
  Slope_400/1 -> Mux/9
  Slope_450/1 -> Mux/10
  Demux/2 -> Acceleration_50/1
  Demux/3 -> Acceleration_100/1
  Demux/4 -> Acceleration_150/1
  Demux/5 -> Acceleration_200/1
  Demux/6 -> Acceleration_250/1
  Demux/7 -> Acceleration_300/1
  Demux/8 -> Acceleration_350/1
  Demux/9 -> Acceleration_400/1
  Demux/10 -> Acceleration_450/1
